simulink model "SIM_EXO_DAL"  (R2021b)
settings: Solver=VariableStepAuto  StartTime=0.0  StopTime=60  FixedStep=0.0001  RelTol=1e-4
undefined symbols (not defined in the file): b, dq, q, X, Y, Z
libraries: sm_lib x47, nesl_utility x7
(part 3 of 25)

== matlab function SIM_EXO_DAL/PID(LGR)/H_Matrix ==
  data: q input; H output
function H = H_Matrix(q)
%#codegen
q1 = q(1);
q2 = q(2);
q3 = q(3);
q4 = q(4);
q5 = q(5);
q6 = q(6);
%    This function was generated by the Symbolic Math Toolbox version 9.0.
%    02-Dec-2021 20:02:35

t2 = cos(q2);
t3 = cos(q4);
t4 = cos(q5);
t5 = cos(q6);
t6 = sin(q2);
t7 = sin(q4);
t8 = sin(q5);
t9 = sin(q6);
t10 = q1+q2;
t11 = q4.*2.0;
t12 = q5.*2.0;
t13 = q6.*2.0;
t30 = 9.007199254740992e+15;
t14 = cos(t12);
t15 = cos(t13);
t16 = t3.^2;
t17 = t4.^2;
t18 = t5.^2;
t19 = sin(t11);
t20 = sin(t12);
t21 = sin(t13);
t22 = cos(t10);
t23 = sin(t10);
t29 = t8.*5.110348748545983e-1;
t31 = t4.*t5.*5.110348748545983e-1;
t32 = t4.*t9.*5.110348748545983e-1;
t33 = t4.*t7.*8.595599785252598e-1;
t34 = t3.*t9.*8.595599785252598e-1;
t35 = t5.*1.33637579258949e-4;
t37 = t3.*t5.*8.595599785252598e-1;
t38 = t9.*7.26350610236655e-5;
t39 = t5.*t7.*t8.*8.595599785252598e-1;
t40 = t7.*t8.*t9.*8.595599785252598e-1;
t41 = t9.*1.744166498897461e-6;
t42 = t5.*1.246862701090643e-6;
t43 = t9.*1.246862701090643e-6;
t44 = t8.*4.20092050615074e-6;
t45 = t5.*3.383302988283333e-6;
t51 = t4.*t9.*3.383302988283333e-6;
t52 = t8.*1.758766830582798e-8;
t53 = t4.*t5.*1.744166498897461e-6;
t54 = t5.*t8.*8.01825475553694e-7;
t55 = t4.*t5.*(-1.246862701090643e-6);
t56 = t4.*t9.*(-1.246862701090643e-6);
t57 = t4.*2.524706033578261e-9;
t58 = t8.*t9.*4.35810366141993e-7;
t59 = t5.*3.146556677756745e-13;
t60 = t8.*3.146556677756745e-13;
t61 = t8.*4.126305279697715e-13;
t62 = t9.*4.126305279697715e-13;
t63 = t4.*t9.*3.146556677756745e-13;
t65 = t4.*t5.*4.126305279697715e-13;
t66 = t5.*t8.*8.4155913e-14;
t67 = t8.*t9.*8.4155913e-14;
t68 = (q3.*t30)./4.503599627370496e+15;
t70 = (q3.*t30)./9.007199254740992e+15;
t78 = t8.*6.829346359246847e-5;
t82 = t3.*5.316841594276996e-5;
t83 = t4.*6.932317328700695e-5;
t84 = t3.*1.166014850920627e-4;
t85 = t3.*t5.*1.148695147579899e-4;
t86 = t8.*3.161026044296245e-5;
t87 = t4.*t9.*6.829346359246847e-5;
t88 = t4.*t7.*1.148695147579899e-4;
t89 = t8.*3.711904932028501e-5;
t90 = t8.*2.146816885134859e-6;
t91 = t8.*3.004073648334264e-7;
t93 = t4.*3.726186752973823e-7;
t94 = t8.*3.726186752973823e-7;
t95 = t4.*t7.*5.316841594276996e-5;
t97 = t4.*3.60334715805357e-7;
t98 = t8.*3.60334715805357e-7;
t99 = t4.*1.153569201933121e-6;
t100 = t7.*t8.*1.166014850920627e-4;
t101 = t3.*2.28624364216682e-6;
t102 = t8.*8.987911871652987e-9;
t103 = t4.*t5.*3.711904932028501e-5;
t104 = t7.*t8.*t9.*1.148695147579899e-4;
t106 = t4.*t7.*6.243419149368285e-5;
t107 = t3.*t9.*6.243419149368285e-5;
t108 = t4.*t5.*8.913299084896471e-7;
t115 = t4.*t9.*1.728985819212562e-6;
t116 = t4.*t5.*6.371903244127231e-7;
t117 = t4.*t9.*6.371903244127231e-7;
t118 = t7.*t8.*1.940301860461398e-6;
t119 = t4.*t7.*3.610943140053254e-6;
t120 = t3.*t5.*2.908151843953269e-6;
t122 = t4.*t7.*5.052847873416058e-7;
t123 = t3.*t5.*1.07175327657342e-6;
t124 = t3.*t9.*1.07175327657342e-6;
t125 = t3.*t9.*1.49921571833678e-6;
t126 = t4.*t7.*6.267441153167058e-7;
t127 = t7.*t8.*6.267441153167058e-7;
t128 = t3.*1.511765579126689e-8;
t129 = t4.*t7.*6.060825118201251e-7;
t131 = t7.*t8.*6.060825118201251e-7;
t134 = t4.*1.290212831914316e-9;
t135 = t8.*1.608000198040319e-13;
t137 = t3.*2.170136264005124e-9;
t140 = t5.*t7.*t8.*6.243419149368285e-5;
t141 = t3.*t4.*t9.*6.892170885479394e-7;
t143 = t7.*t8.*t9.*2.908151843953269e-6;
t144 = t5.*t7.*t8.*1.07175327657342e-6;
t146 = t7.*t8.*t9.*1.07175327657342e-6;
t147 = t5.*t7.*t8.*1.49921571833678e-6;
t149 = t4.*t7.*1.511765579126689e-8;
t150 = t4.*t9.*1.608000198040319e-13;
t153 = t7.*t8.*2.170136264005124e-9;
t154 = t3.*t8.*(-1.511765579126689e-8);
t157 = t3.*t4.*t5.*3.746051489620971e-7;
t158 = t4.*t5.*7.16776774470491e-12;
t159 = t4.*t9.*7.16776774470491e-12;
t160 = t8.*2.10868590222219e-13;
t161 = t3.*t5.*2.7046541903611e-13;
t162 = t4.*t7.*2.7046541903611e-13;
t164 = t3.*t5.*1.205617579517561e-11;
t165 = t3.*t9.*1.205617579517561e-11;
t167 = t4.*t7.*3.546806877605634e-13;
t168 = t3.*t9.*3.546806877605634e-13;
t169 = t4.*t5.*2.10868590222219e-13;
t172 = t7.*t8.*t9.*2.7046541903611e-13;
t173 = t5.*t7.*t8.*1.205617579517561e-11;
t174 = t7.*t8.*t9.*1.205617579517561e-11;
t177 = t5.*t7.*t8.*3.546806877605634e-13;
t180 = t3.*t8.*t9.*(-3.546806877605634e-13);
t192 = t3.*2.625549359694895e-3;
t193 = t4.*1.560969940408669e-3;
t194 = t8.*1.560969940408669e-3;
t195 = t6.*t8.*1.324388487819695e-2;
t196 = t2.*t8.*5.463144604697158e-2;
t202 = t4.*t7.*2.625549359694895e-3;
t204 = t7.*t8.*2.625549359694895e-3;
t207 = t4.*t6.*t7.*2.227619671697157e-2;
t208 = t7.*5.363539617571206e-4;
t209 = t3.*t5.*(-2.625549359694895e-3);
t210 = t4.*t5.*(-1.560969940408669e-3);
t211 = t4.*t9.*(-1.560969940408669e-3);
t217 = t2.*t4.*t7.*9.189001945180305e-2;
t218 = t5.*1.184846851663018e-6;
t223 = t7.*3.050168925520967e-6;
t226 = t7.*6.689201101650821e-6;
t230 = t3.*t4.*5.363539617571206e-4;
t231 = t3.*t8.*5.363539617571206e-4;
t233 = t3.*t9.*6.589841321991422e-6;
t237 = t3.*t4.*3.050168925520967e-6;
t240 = t3.*t8.*6.689201101650821e-6;
t246 = t3.*t8.*1.545129867076994e-8;
t247 = t3.*t4.*t9.*7.044279371874937e-7;
t248 = t9.*6.439911875946239e-7;
t249 = t3.*t5.*3.581728501918121e-6;
t255 = t5.*t7.*t8.*6.589841321991422e-6;
t269 = t3.*t7.*t8.*t9.*4.188040994443703e-7;
t270 = t3.*2.783427048984746e-6;
t271 = t4.*t5.*t7.*t8.*1.408855874374987e-6;
t272 = t3.*t4.*t5.*t9.*1.440030993265091e-6;
t273 = t7.*t8.*t9.*3.581728501918121e-6;
t275 = t3.*t4.*t7.*9.186272837068685e-9;
t280 = t3.*t4.*3.476977846858022e-8;
t281 = t3.*t8.*3.476977846858022e-8;
t282 = t3.*t4.*t5.*3.828725908394669e-7;
t286 = t3.*t5.*t7.*t8.*t9.*8.561427670149984e-7;
t294 = t3.*t5.*t7.*t8.*2.276295446893622e-7;
t302 = t7.*t8.*5.200343311959535e-6;
t303 = t7.*t9.*2.764345231392299e-13;
t306 = t4.*t5.*t7.*t8.*t9.*2.190813206274814e-6;
t308 = t3.*t4.*1.093188572509221e-6;
t311 = t4.*t7.*t8.*t9.*7.657451816789338e-7;
t320 = t3.*t5.*t8.*2.764345231392299e-13;
t328 = t4.*t8.*t9.*3.006136635626675e-13;
t332 = t5.*t7.*3.625084017661248e-13;
t335 = t3.*t7.*t8.*6.499342678834474e-7;
t341 = t3.*t4.*t5.*t7.*1.643488359943407e-13;
t345 = t3.*t8.*t9.*3.625084017661248e-13;
t346 = t4.*t7.*t8.*5.185406908527248e-7;
t348 = t4.*t5.*t8.*3.94216241479634e-13;
t350 = t3.*t4.*t7.*t9.*2.155224072299545e-13;
t360 = t4.*t7.*6.689200410011394e-6;
t379 = t8.*2.086042441322004e-7;
t384 = t8.*1.133811468776912e-7;
t386 = t4.*t9.*2.086042441322004e-7;
t388 = t2.*t4.*t5.*1.769880715106441e-6;
t389 = t4.*t6.*t9.*1.769880715106441e-6;
t390 = t5.*t6.*t8.*1.769880715106441e-6;
t391 = t3.*4.911624408131596e-10;
t392 = t4.*t5.*1.133811468776912e-7;
t394 = t3.*t5.*3.508720606545093e-7;
t397 = t4.*t7.*3.508720606545093e-7;
t398 = t7.*t9.*3.508720606545093e-7;
t399 = t2.*t7.*4.167215943261981e-9;
t400 = t3.*t6.*4.167215943261981e-9;
t401 = t6.*t7.*t9.*2.976937004352228e-6;
t402 = t4.*t5.*1.209061939415321e-5;
t405 = t2.*t4.*t9.*7.30081420113316e-6;
t406 = t2.*t5.*t8.*7.30081420113316e-6;
t407 = t4.*t5.*t6.*7.30081420113316e-6;
t410 = t2.*t3.*t9.*2.976937004352228e-6;
t411 = t3.*t5.*t6.*2.976937004352228e-6;
t414 = t8.*1.646190906295504e-7;
t415 = t2.*t3.*t5.*1.22799597575967e-5;
t417 = t2.*t7.*t9.*1.22799597575967e-5;
t418 = t3.*t6.*t9.*1.22799597575967e-5;
t422 = t3.*t9.*2.033640570959539e-5;
t423 = t4.*t7.*1.907069379620846e-7;
t424 = t3.*t9.*1.907069379620846e-7;
t425 = t5.*t7.*1.907069379620846e-7;
t428 = t6.*t8.*t9.*9.619703863182361e-7;
t429 = t2.*t4.*1.396693317797299e-6;
t430 = t6.*t8.*1.396693317797299e-6;
t431 = t2.*t4.*t5.*3.96815841743287e-6;
t432 = t2.*t8.*t9.*3.96815841743287e-6;
t433 = t4.*t6.*t9.*3.96815841743287e-6;
t434 = t2.*t3.*t5.*1.618032907912407e-6;
t437 = t2.*t3.*1.718989821069714e-8;
t438 = t3.*t6.*t9.*1.618032907912407e-6;
t439 = t5.*t6.*t7.*1.618032907912407e-6;
t440 = t6.*t7.*1.718989821069714e-8;
t441 = t7.*t8.*t9.*(-3.508720606545093e-7);
t443 = t2.*t5.*t7.*t8.*2.976937004352228e-6;
t445 = t4.*t5.*t6.*t7.*2.976937004352228e-6;
t446 = t2.*t4.*t9.*9.619703863182361e-7;
t447 = t4.*t5.*t6.*9.619703863182361e-7;
t449 = t4.*t9.*6.571526380364474e-6;
t451 = t3.*t5.*1.105329861487718e-5;
t453 = t2.*t4.*t5.*t7.*1.22799597575967e-5;
t457 = t5.*t6.*t7.*t8.*1.22799597575967e-5;
t461 = t7.*4.452917654948397e-7;
t462 = t5.*t7.*t8.*2.033640570959539e-5;
t466 = t2.*t8.*5.761404326386517e-6;
t467 = t4.*t6.*5.761404326386517e-6;
t469 = t3.*t5.*t6.*t8.*(-2.976937004352228e-6);
t471 = t2.*t3.*t9.*6.674437170347525e-6;
t472 = t2.*t5.*t7.*6.674437170347525e-6;
t473 = t3.*t5.*t6.*6.674437170347525e-6;
t474 = t4.*9.541257312828922e-6;
t476 = t3.*t8.*2.768890910755245e-7;
t477 = t4.*t7.*2.768890910755245e-7;
t478 = t2.*t3.*3.778031034908185e-6;
t479 = t2.*t7.*t8.*t9.*(-1.22799597575967e-5);
t481 = t6.*t7.*3.778031034908185e-6;
t482 = t2.*t7.*t8.*t9.*1.618032907912407e-6;
t484 = t4.*t6.*t7.*t9.*1.618032907912407e-6;
t488 = t7.*t8.*t9.*1.105329861487718e-5;
t490 = t2.*t7.*t8.*2.349236299369594e-6;
t491 = t3.*t6.*t8.*2.349236299369594e-6;
t492 = t4.*t6.*t7.*2.349236299369594e-6;
t494 = t3.*t6.*t8.*t9.*(-1.618032907912407e-6);
t496 = t5.*t6.*t7.*t8.*(-1.618032907912407e-6);
t497 = t2.*t7.*1.558449809444963e-5;
t498 = t3.*t6.*1.558449809444963e-5;
t500 = t2.*t4.*t7.*t9.*6.674437170347525e-6;
t502 = t6.*t7.*t8.*t9.*6.674437170347525e-6;
t503 = t3.*2.010604972694953e-5;
t511 = t4.*t5.*2.189414175010785e-14;
t512 = t4.*t9.*2.189414175010785e-14;
t513 = t7.*t8.*1.604838208596364e-5;
t514 = t2.*t3.*t8.*9.690674399615435e-6;
t515 = t2.*t4.*t7.*9.690674399615435e-6;
t516 = t6.*t7.*t8.*9.690674399615435e-6;
t517 = t7.*6.664488561844862e-7;
t519 = t3.*t5.*3.682591724861488e-14;
t521 = t3.*t9.*3.682591724861488e-14;
t524 = t5.*t7.*t8.*3.682591724861488e-14;
t525 = t7.*t8.*t9.*3.682591724861488e-14;
t526 = t4.*2.11749498538388e-7;
t534 = t2.*t8.*1.796566294495167e-6;
t535 = t4.*t6.*1.796566294495167e-6;
t539 = t2.*t4.*7.410893064247368e-6;
t540 = t6.*t8.*7.410893064247368e-6;
t542 = t3.*t4.*3.561623743745041e-7;
t543 = t7.*t8.*3.561623743745041e-7;
t544 = t8.*1.227291709418896e-5;
t545 = t2.*t4.*t7.*3.021822113324163e-6;
t546 = t3.*t4.*t6.*3.021822113324163e-6;
t547 = t6.*t7.*t8.*3.021822113324163e-6;
t553 = t4.*t7.*2.06430301981345e-5;
t556 = t2.*t3.*t4.*1.246511225866906e-5;
t557 = t2.*t7.*t8.*1.246511225866906e-5;
t558 = t4.*t6.*t7.*1.246511225866906e-5;
t593 = t2.*1.410504133294943e-4;
t596 = t6.*4.897880306001738e-4;
t24 = t23.*7.742227997977903e+15;
t25 = t22.*4.602992943936994e+15;
t26 = t23.*4.602992943936994e+15;
t27 = t22.*7.742227997977903e+15;
t36 = -t31;
t46 = -t40;
t48 = t4.*t42;
t49 = t4.*t43;
t64 = -t62;
t69 = sin(t68);
t71 = cos(t70);
t72 = sin(t70);
t92 = -t83;
t96 = -t90;
t105 = -t93;
t109 = -t97;
t110 = -t98;
t111 = -t99;
t112 = -t102;
t113 = -t103;
t114 = -t104;
t121 = t29+t33;
t130 = -t116;
t132 = -t117;
t133 = -t119;
t136 = -t123;
t138 = -t125;
t139 = -t128;
t142 = -t129;
t145 = -t134;
t148 = t8.*t128;
t151 = -t143;
t152 = -t147;
t155 = -t149;
t156 = -t150;
t163 = -t157;
t166 = -t161;
t170 = -t165;
t171 = t8.*t161;
t175 = -t169;
t176 = t8.*t168;
t178 = -t173;
t179 = -t174;
t181 = t52+t57;
t182 = t20.*3.726186322907759e-7;
t197 = -t193;
t200 = -t195;
t201 = t5.*t192;
t203 = t9.*t192;
t205 = t5.*t193;
t206 = t9.*t193;
t219 = -t207;
t221 = t5.*t204;
t222 = t9.*t204;
t224 = t18.*4.280713835074992e-7;
t229 = t21.*3.256264776948168e-7;
t251 = t5.*t16.*4.188040994443703e-7;
t253 = t5.*t17.*7.660427522186475e-7;
t257 = t9.*t16.*2.276295446893622e-7;
t258 = t16.*t18.*8.561427670149984e-7;
t260 = t19.*4.420145378913349e-10;
t261 = -t247;
t262 = -t249;
t268 = t5.*t9.*t16.*1.302505910779267e-6;
t276 = t17.*t18.*7.829937223708732e-7;
t277 = t5.*t9.*t17.*1.191219491402018e-6;
t278 = t3.*t4.*t18.*2.190813206274814e-6;
t287 = -t269;
t288 = -t270;
t289 = -t271;
t290 = t9.*t17.*4.163616429052617e-7;
t291 = -t272;
t292 = -t275;
t297 = -t281;
t298 = t3.*t7.*t8.*t18.*1.302505910779267e-6;
t305 = -t286;
t309 = t4.*t7.*t8.*t18.*1.440030993265091e-6;
t315 = -t306;
t316 = -t308;
t321 = -t311;
t322 = t5.*t16.*t17.*(-4.188040994443703e-7);
t324 = t5.*t9.*t16.*t17.*6.512529553896337e-7;
t325 = t16.*1.035461175802946e-6;
t326 = t9.*t16.*t17.*(-2.276295446893622e-7);
t327 = t16.*t17.*t18.*(-4.280713835074992e-7);
t329 = t17.*2.81948171692439e-7;
t331 = -t320;
t338 = t7.*t9.*t17.*5.528690462784599e-13;
t343 = -t335;
t347 = t4.*t8.*t9.*t16.*1.643488359943407e-13;
t349 = t16.*t17.*1.54144203823673e-7;
t351 = -t350;
t352 = t5.*t7.*t17.*7.250168035322496e-13;
t353 = t4.*t5.*t8.*t16.*2.155224072299545e-13;
t355 = t35+t38+4.36041e-5;
t362 = -t360;
t363 = t20.*3.483029800032151e-7;
t364 = t43+t45+8.01825475553694e-7;
t365 = t7.*t17.*1.281152254279884e-6;
t368 = t41+t42+4.35810366141993e-7;
t371 = t4.*t8.*t16.*3.808422322424164e-7;
t387 = t5.*t379;
t393 = t9.*t384;
t395 = -t389;
t396 = -t390;
t404 = -t392;
t409 = -t398;
t412 = -t399;
t413 = -t400;
t419 = t8.*t394;
t420 = t5.*t397;
t421 = t8.*t398;
t426 = -t410;
t427 = -t411;
t435 = -t417;
t436 = -t418;
t442 = -t422;
t444 = t8.*t411;
t448 = t8.*t401;
t450 = -t428;
t452 = t8.*t415;
t454 = -t430;
t455 = -t431;
t456 = t8.*t417;
t458 = -t438;
t459 = -t439;
t460 = -t440;
t463 = t8.*t424;
t464 = t9.*t423;
t465 = t8.*t425;
t468 = -t443;
t470 = -t445;
t480 = -t457;
t483 = t8.*t438;
t485 = t8.*t439;
t486 = -t462;
t489 = -t481;
t493 = -t482;
t495 = -t484;
t499 = t8.*t471;
t501 = t8.*t472;
t505 = -t488;
t506 = -t490;
t507 = -t491;
t508 = -t492;
t509 = -t502;
t518 = -t513;
t520 = -t516;
t522 = -t517;
t523 = -t521;
t531 = -t524;
t532 = -t525;
t533 = -t526;
t541 = -t539;
t548 = -t542;
t554 = -t547;
t560 = -t556;
t712 = t51+t55+t60+t67;
t736 = t53+t56+t61+t66;
t1090 = t44+t54+t58+t63+t65;
t28 = -t26;
t47 = t24+t25;
t73 = t71.^2;
t74 = t3.*t71;
t75 = t7.*t71;
t76 = t71-1.0;
t183 = t71.*2.118754404193375e+31;
t184 = -t182;
t186 = t59+t64;
t189 = t4.*t71.*5.157359871151559e-3;
t232 = -t224;
t234 = -t229;
t267 = -t253;
t295 = -t276;
t296 = -t277;
t307 = -t290;
t312 = t17.*t251;
t317 = t17.*t257;
t318 = t16.*t17.*t224;
t319 = -t309;
t336 = -t324;
t337 = -t325;
t340 = t3.*t30.*t72.*4.602992943936994e+15;
t344 = -t338;
t354 = -t352;
t356 = t34+t36+t39;
t357 = t32+t37+t46;
t361 = t3.*t8.*t30.*t72.*6.661338147750939e-19;
t366 = -t363;
t369 = t71.*7.38843356682345e-1;
t370 = t71.*2.61156643317655e-1;
t372 = t71.*4.392651260556773e-1;
t373 = t71.*4.931128922368695e-2;
t374 = -t371;
t377 = t30.*t72.*8.001214128951626e+33;
t381 = t4.*t30.*t72.*8.368294830410569e+32;
t382 = t7.*t8.*t30.*t72.*4.97520895370488e+32;
t383 = t4.*t71.*1.511765579126689e-8;
t403 = t4.*t16.*t71.*3.023531158253378e-8;
t408 = t16.*t71.*2.909656073620116e-9;
t487 = -t7.*t30.*t72.*(t26-t27);
t510 = t7.*t30.*t72.*(t26-t27);
t527 = t3.*t30.*t72.*5.673626844500105e-17;
t528 = t7.*t30.*t72.*5.673626844500105e-17;
t529 = t4.*t30.*t72.*9.543032792050485e-17;
t530 = t8.*t30.*t72.*9.543032792050485e-17;
t538 = t3.*t30.*t72.*3.404176106700063e-19;
t549 = t5.*t8.*t30.*t72.*5.725819675230291e-19;
t550 = t8.*t9.*t30.*t72.*5.725819675230291e-19;
t551 = t4.*t5.*t7.*t30.*t72.*3.404176106700063e-19;
t552 = t4.*t7.*t9.*t30.*t72.*3.404176106700063e-19;
t561 = t2.*t8.*t71.*2.227619671697157e-2;
t562 = t4.*t71.*5.088811214040866e-2;
t563 = t8.*t71.*5.088811214040866e-2;
t565 = t6.*t8.*t71.*9.189001945180305e-2;
t588 = t2.*t71.*4.472183499114333e-13;
t603 = t6.*t71.*1.844789907123413e-12;
t614 = t71.*1.454432002254732e-9;
t653 = t3.*t30.*t72.*(t26-t27).*(-1.232595164407831e-32);
t666 = t7.*t30.*t72.*9.827649182848514e-18;
H = ft_1({t100,t101,t102,t105,t106,t107,t108,t109,t1090,t110,t111,t112,t113,t114,t115,t118,t119,t120,t121,t122,t124,t126,t127,t130,t131,t132,t133,t134,t135,t136,t137,t138,t139,t14,t140,t141,t142,t144,t145,t146,t149,t15,t150,t151,t152,t153,t154,t155,t156,t158,t159,t16,t160,t161,t162,t163,t164,t166,t167,t168,t169,t17,t170,t171,t172,t175,t177,t178,t179,t18,t180,t181,t183,t184,t186,t189,t19,t192,t194,t196,t197,t2,t20,t200,t202,t203,t204,t208,t209,t21,t210,t211,t217,t218,t219,t22,t221,t222,t223,t226,t23,t230,t231,t232,t233,t234,t237,t240,t246,t247,t248,t251,t253,t255,t257,t258,t26,t260,t261,t262,t267,t268,t27,t271,t272,t273,t276,t277,t278,t28,t280,t282,t287,t288,t289,t290,t291,t292,t294,t295,t296,t297,t298,t3,t30,t302,t303,t305,t306,t307,t308,t309,t311,t315,t316,t319,t320,t321,t322,t326,t327,t328,t329,t331,t332,t336,t337,t338,t340,t341,t343,t344,t345,t346,t347,t348,t349,t35,t351,t352,t353,t354,t355,t356,t357,t361,t362,t364,t365,t366,t368,t369,t370,t372,t373,t374,t377,t379,t38,t381,t382,t383,t384,t386,t387,t388,t390,t391,t393,t394,t395,t396,t397,t4,t401,t402,t403,t404,t405,t406,t407,t408,t409,t41,t412,t413,t414,t415,t419,t42,t420,t423,t424,t425,t426,t427,t428,t429,t43,t430,t432,t433,t434,t435,t436,t437,t441,t442,t446,t447,t448,t449,t45,t450,t451,t452,t453,t454,t455,t458,t459,t460,t461,t463,t464,t465,t466,t467,t468,t469,t47,t470,t471,t472,t473,t474,t476,t477,t478,t479,t480,t486,t489,t493,t494,t495,t496,t497,t498,t499,t5,t500,t501,t503,t505,t506,t507,t508,t509,t510,t511,t512,t514,t515,t518,t519,t52,t520,t521,t522,t523,t524,t527,t528,t529,t530,t531,t532,t533,t534,t535,t538,t539,t540,t541,t543,t544,t545,t546,t548,t549,t550,t551,t552,t553,t554,t557,t558,t560,t561,t562,t563,t565,t588,t59,t593,t596,t6,t603,t61,t614,t62,t653,t666,t69,t7,t71,t712,t72,t73,t736,t74,t75,t76,t78,t8,t82,t84,t85,t86,t87,t88,t89,t9,t90,t91,t92,t94,t95,t96});
end
function H = ft_1(ct)
t100 = ct{1};
t101 = ct{2};
t102 = ct{3};
t105 = ct{4};
t106 = ct{5};
t107 = ct{6};
t108 = ct{7};
t109 = ct{8};
t1090 = ct{9};
t110 = ct{10};
t111 = ct{11};
t112 = ct{12};
t113 = ct{13};
t114 = ct{14};
t115 = ct{15};
t118 = ct{16};
t119 = ct{17};
t120 = ct{18};
t121 = ct{19};
t122 = ct{20};
t124 = ct{21};
t126 = ct{22};
t127 = ct{23};
t130 = ct{24};
t131 = ct{25};
t132 = ct{26};
t133 = ct{27};
t134 = ct{28};
t135 = ct{29};
t136 = ct{30};
t137 = ct{31};
t138 = ct{32};
t139 = ct{33};
t14 = ct{34};
t140 = ct{35};
t141 = ct{36};
t142 = ct{37};
t144 = ct{38};
t145 = ct{39};
t146 = ct{40};
t149 = ct{41};
t15 = ct{42};
t150 = ct{43};
t151 = ct{44};
t152 = ct{45};
t153 = ct{46};
t154 = ct{47};
t155 = ct{48};
t156 = ct{49};
t158 = ct{50};
t159 = ct{51};
t16 = ct{52};
t160 = ct{53};
t161 = ct{54};
t162 = ct{55};
t163 = ct{56};
t164 = ct{57};
t166 = ct{58};
t167 = ct{59};
t168 = ct{60};
t169 = ct{61};
t17 = ct{62};
t170 = ct{63};
t171 = ct{64};
t172 = ct{65};
t175 = ct{66};
t177 = ct{67};
t178 = ct{68};
t179 = ct{69};
t18 = ct{70};
t180 = ct{71};
t181 = ct{72};
t183 = ct{73};
t184 = ct{74};
t186 = ct{75};
t189 = ct{76};
t19 = ct{77};
t192 = ct{78};
t194 = ct{79};
t196 = ct{80};
t197 = ct{81};
t2 = ct{82};
t20 = ct{83};
t200 = ct{84};
t202 = ct{85};
t203 = ct{86};
t204 = ct{87};
t208 = ct{88};
t209 = ct{89};
t21 = ct{90};
t210 = ct{91};
t211 = ct{92};
t217 = ct{93};
t218 = ct{94};
t219 = ct{95};
t22 = ct{96};
t221 = ct{97};
t222 = ct{98};
t223 = ct{99};
t226 = ct{100};
t23 = ct{101};
t230 = ct{102};
t231 = ct{103};
t232 = ct{104};
t233 = ct{105};
t234 = ct{106};
t237 = ct{107};
t240 = ct{108};
t246 = ct{109};
t247 = ct{110};
t248 = ct{111};
t251 = ct{112};
t253 = ct{113};
t255 = ct{114};
t257 = ct{115};
t258 = ct{116};
t26 = ct{117};
t260 = ct{118};
t261 = ct{119};
t262 = ct{120};
t267 = ct{121};
t268 = ct{122};
t27 = ct{123};
t271 = ct{124};
t272 = ct{125};
t273 = ct{126};
t276 = ct{127};
t277 = ct{128};
t278 = ct{129};
t28 = ct{130};
t280 = ct{131};
t282 = ct{132};
t287 = ct{133};
t288 = ct{134};
t289 = ct{135};
t290 = ct{136};
t291 = ct{137};
t292 = ct{138};
t294 = ct{139};
t295 = ct{140};
t296 = ct{141};
t297 = ct{142};
t298 = ct{143};
t3 = ct{144};
t30 = ct{145};
t302 = ct{146};
t303 = ct{147};
t305 = ct{148};
t306 = ct{149};
t307 = ct{150};
t308 = ct{151};
t309 = ct{152};
t311 = ct{153};
t315 = ct{154};
t316 = ct{155};
t319 = ct{156};
t320 = ct{157};
t321 = ct{158};
t322 = ct{159};
t326 = ct{160};
t327 = ct{161};
t328 = ct{162};
t329 = ct{163};
t331 = ct{164};
t332 = ct{165};
t336 = ct{166};
t337 = ct{167};
t338 = ct{168};
t340 = ct{169};
t341 = ct{170};
t343 = ct{171};
t344 = ct{172};
t345 = ct{173};
t346 = ct{174};
t347 = ct{175};
t348 = ct{176};
t349 = ct{177};
t35 = ct{178};
t351 = ct{179};
t352 = ct{180};
t353 = ct{181};
t354 = ct{182};
t355 = ct{183};
t356 = ct{184};
t357 = ct{185};
t361 = ct{186};
t362 = ct{187};
t364 = ct{188};
t365 = ct{189};
t366 = ct{190};
t368 = ct{191};
t369 = ct{192};
t370 = ct{193};
t372 = ct{194};
t373 = ct{195};
t374 = ct{196};
t377 = ct{197};
t379 = ct{198};
t38 = ct{199};
t381 = ct{200};
t382 = ct{201};
t383 = ct{202};
t384 = ct{203};
t386 = ct{204};
t387 = ct{205};
t388 = ct{206};
t390 = ct{207};
t391 = ct{208};
t393 = ct{209};
t394 = ct{210};
t395 = ct{211};
t396 = ct{212};
t397 = ct{213};
t4 = ct{214};
t401 = ct{215};
t402 = ct{216};
t403 = ct{217};
t404 = ct{218};
t405 = ct{219};
t406 = ct{220};
t407 = ct{221};
t408 = ct{222};
t409 = ct{223};
t41 = ct{224};
t412 = ct{225};
t413 = ct{226};
t414 = ct{227};
t415 = ct{228};
t419 = ct{229};
t42 = ct{230};
t420 = ct{231};
t423 = ct{232};
t424 = ct{233};
t425 = ct{234};
t426 = ct{235};
t427 = ct{236};
t428 = ct{237};
t429 = ct{238};
t43 = ct{239};
t430 = ct{240};
t432 = ct{241};
t433 = ct{242};
t434 = ct{243};
t435 = ct{244};
t436 = ct{245};
t437 = ct{246};
t441 = ct{247};
t442 = ct{248};
t446 = ct{249};
t447 = ct{250};
t448 = ct{251};
t449 = ct{252};
t45 = ct{253};
t450 = ct{254};
t451 = ct{255};
t452 = ct{256};
t453 = ct{257};
t454 = ct{258};
t455 = ct{259};
t458 = ct{260};
t459 = ct{261};
t460 = ct{262};
t461 = ct{263};
t463 = ct{264};
t464 = ct{265};
t465 = ct{266};
t466 = ct{267};
t467 = ct{268};
t468 = ct{269};
t469 = ct{270};
t47 = ct{271};
t470 = ct{272};
t471 = ct{273};
t472 = ct{274};
t473 = ct{275};
t474 = ct{276};
t476 = ct{277};
t477 = ct{278};
t478 = ct{279};
t479 = ct{280};
t480 = ct{281};
t486 = ct{282};
t489 = ct{283};
t493 = ct{284};
t494 = ct{285};
t495 = ct{286};
t496 = ct{287};
t497 = ct{288};
t498 = ct{289};
t499 = ct{290};
t5 = ct{291};
t500 = ct{292};
t501 = ct{293};
t503 = ct{294};
t505 = ct{295};
t506 = ct{296};
t507 = ct{297};
t508 = ct{298};
t509 = ct{299};
t510 = ct{300};
t511 = ct{301};
t512 = ct{302};
t514 = ct{303};
t515 = ct{304};
t518 = ct{305};
t519 = ct{306};
t52 = ct{307};
t520 = ct{308};
t521 = ct{309};
t522 = ct{310};
t523 = ct{311};
t524 = ct{312};
t527 = ct{313};
t528 = ct{314};
t529 = ct{315};
t530 = ct{316};
t531 = ct{317};
t532 = ct{318};
t533 = ct{319};
t534 = ct{320};
t535 = ct{321};
t538 = ct{322};
t539 = ct{323};
t540 = ct{324};
t541 = ct{325};
t543 = ct{326};
t544 = ct{327};
t545 = ct{328};
t546 = ct{329};
t548 = ct{330};
t549 = ct{331};
t550 = ct{332};
t551 = ct{333};
t552 = ct{334};
t553 = ct{335};
t554 = ct{336};
t557 = ct{337};
t558 = ct{338};
t560 = ct{339};
t561 = ct{340};
t562 = ct{341};
t563 = ct{342};
t565 = ct{343};
t588 = ct{344};
t59 = ct{345};
t593 = ct{346};
t596 = ct{347};
t6 = ct{348};
t603 = ct{349};
t61 = ct{350};
t614 = ct{351};
t62 = ct{352};
t653 = ct{353};
t666 = ct{354};
t69 = ct{355};
t7 = ct{356};
t71 = ct{357};
t712 = ct{358};
t72 = ct{359};
t73 = ct{360};
t736 = ct{361};
t74 = ct{362};
t75 = ct{363};
t76 = ct{364};
t78 = ct{365};
t8 = ct{366};
t82 = ct{367};
t84 = ct{368};
t85 = ct{369};
t86 = ct{370};
t87 = ct{371};
t88 = ct{372};
t89 = ct{373};
t9 = ct{374};
t90 = ct{375};
t91 = ct{376};
t92 = ct{377};
t94 = ct{378};
t95 = ct{379};
t96 = ct{380};
t668 = t8.*t30.*t72.*4.008952214699383e-22;
t670 = t2.*t3.*t4.*t30.*t72.*2.877233365226343e-18;
t671 = t3.*t30.*t72.*4.549258542705501e-23;
t672 = t3.*t4.*t6.*t30.*t72.*1.186867907736671e-17;
t674 = t3.*t4.*t30.*t72.*9.827649182848514e-18;
t676 = t3.*t8.*t30.*t72.*9.827649182848514e-18;
t679 = t5.*t30.*t72.*1.530369361342075e-22;
t681 = t7.*t9.*t30.*t72.*(-9.827649182848514e-18);
t682 = t3.*t5.*t30.*t72.*9.098517085411002e-23;
t685 = t3.*t30.*t72.*2.472625392454631e-23;
t686 = t3.*t5.*t9.*t30.*t72.*1.414846738462756e-22;
t687 = t8.*t30.*t72.*1.678396953782234e-24;
t688 = t3.*t9.*t30.*t72.*4.945250784909262e-23;
t689 = t9.*t30.*t72.*8.317905230417136e-23;
t691 = t4.*t5.*t7.*t30.*t72.*4.549258542705501e-23;
t692 = t7.*t8.*t9.*t30.*t72.*4.549258542705501e-23;
t693 = t3.*t18.*t30.*t72.*9.299848787979342e-23;
t694 = t4.*t9.*t30.*t72.*7.651846806710377e-23;
t695 = t5.*t8.*t30.*t72.*7.651846806710377e-23;
t696 = t3.*t8.*t30.*t72.*9.978586703210931e-25;
t697 = t4.*t7.*t30.*t72.*9.978586703210931e-25;
t700 = t4.*t18.*t30.*t72.*2.379770328738529e-22;
t701 = t3.*t4.*t9.*t30.*t72.*(-4.549258542705501e-23);
t705 = t4.*t5.*t9.*t30.*t72.*1.564233326885588e-22;
t707 = t5.*t17.*t30.*t72.*(-1.530369361342075e-22);
t708 = t3.*t4.*t5.*t9.*t30.*t72.*9.299848787979342e-23;
t709 = t5.*t7.*t8.*t9.*t30.*t72.*9.299848787979342e-23;
t710 = t4.*t5.*t30.*t72.*4.158952615208568e-23;
t711 = t8.*t9.*t30.*t72.*4.158952615208568e-23;
t713 = t4.*t5.*t7.*t8.*t30.*t72.*9.098517085411002e-23;
t714 = t3.*t4.*t18.*t30.*t72.*1.414846738462756e-22;
t715 = t7.*t8.*t18.*t30.*t72.*1.414846738462756e-22;
t717 = t7.*t9.*t30.*t72.*1.785238843466173e-29;
t720 = t8.*t30.*t72.*3.002769355787804e-29;
t722 = t4.*t7.*t9.*t30.*t72.*2.472625392454631e-23;
t723 = t5.*t7.*t8.*t30.*t72.*2.472625392454631e-23;
t724 = t5.*t9.*t17.*t30.*t72.*2.379770328738529e-22;
t726 = t17.*t18.*t30.*t72.*1.564233326885588e-22;
t727 = t4.*t5.*t7.*t8.*t9.*t30.*t72.*1.414846738462756e-22;
t729 = t4.*t7.*t8.*t9.*t30.*t72.*4.945250784909262e-23;
t732 = t4.*t7.*t8.*t18.*t30.*t72.*9.299848787979342e-23;
t733 = t4.*t30.*t72.*1.187475829122392e-22;
t735 = t3.*t4.*t30.*t72.*7.059909452387201e-23;
t738 = t7.*t8.*t30.*t72.*7.059909452387201e-23;
t744 = t30.*t72.*8.730562784510963e-22;
t748 = t9.*t17.*t30.*t72.*(-8.317905230417136e-23);
t749 = t3.*t5.*t8.*t30.*t72.*1.785238843466173e-29;
t750 = t4.*t5.*t7.*t30.*t72.*1.785238843466173e-29;
t752 = t8.*t30.*t72.*3.937746659416635e-29;
t753 = t4.*t8.*t9.*t30.*t72.*6.005538711575609e-29;
t754 = t5.*t8.*t30.*t72.*(-3.002769355787804e-29);
t755 = t30.*t69.*9.59842590807046e-26;
t758 = t17.*t30.*t72.*5.632647031707275e-23;
t760 = t3.*t30.*t72.*2.647073057000717e-22;
t761 = t4.*t5.*t71.*7.017441213090186e-7;
t764 = t7.*t9.*t17.*t30.*t72.*3.570477686932346e-29;
t766 = t5.*t7.*t30.*t72.*2.341111640349547e-29;
t772 = t4.*t7.*t8.*t30.*t72.*3.34878210114812e-23;
t773 = t8.*t71.*6.800564119502148e-6;
t780 = t4.*t9.*t71.*3.814138759241691e-7;
t782 = t2.*t4.*t9.*t71.*2.976937004352228e-6;
t783 = t2.*t5.*t8.*t71.*2.976937004352228e-6;
t784 = t4.*t5.*t6.*t71.*2.976937004352228e-6;
t785 = t5.*t8.*t30.*t72.*8.031026374039477e-30;
t786 = t8.*t9.*t30.*t72.*8.031026374039477e-30;
t789 = t4.*t5.*t8.*t30.*t72.*7.875493318833269e-29;
t791 = t3.*t8.*t9.*t30.*t72.*2.341111640349547e-29;
t792 = t4.*t7.*t9.*t30.*t72.*2.341111640349547e-29;
t798 = t8.*t71.*3.696261130697717e-6;
t799 = t5.*t7.*t17.*t30.*t72.*4.682223280699094e-29;
t804 = t4.*t9.*t71.*6.800564119502148e-6;
t817 = t2.*t4.*t5.*t71.*1.22799597575967e-5;
t818 = t4.*t5.*t7.*t30.*t72.*4.774692471202153e-30;
t821 = t4.*t7.*t9.*t30.*t72.*4.774692471202153e-30;
t824 = t4.*t6.*t9.*t71.*1.22799597575967e-5;
t825 = t5.*t6.*t8.*t71.*1.22799597575967e-5;
t834 = t5.*t8.*t71.*(-6.800564119502148e-6);
t837 = t4.*t71.*5.537781821510491e-7;
t843 = t2.*t4.*t5.*t71.*1.618032907912407e-6;
t847 = t2.*t8.*t9.*t71.*1.618032907912407e-6;
t848 = t4.*t6.*t9.*t71.*1.618032907912407e-6;
t853 = t2.*t4.*t9.*t71.*6.674437170347525e-6;
t854 = t4.*t5.*t6.*t71.*6.674437170347525e-6;
t855 = t6.*t8.*t9.*t71.*6.674437170347525e-6;
t867 = t4.*t5.*t71.*3.696261130697717e-6;
t870 = t2.*t8.*t71.*2.349236299369594e-6;
t871 = t4.*t6.*t71.*2.349236299369594e-6;
t894 = t8.*t9.*t71.*(-3.696261130697717e-6);
t899 = t2.*t4.*t71.*9.690674399615435e-6;
t902 = t6.*t8.*t71.*9.690674399615435e-6;
t910 = t8.*t71.*5.366634249353632e-6;
t915 = t7.*t17.*t30.*t72.*8.273795699471084e-23;
t917 = t4.*t8.*t30.*t72.*1.391651334125335e-22;
t923 = t4.*t5.*t71.*7.137559230037459e-13;
t924 = t4.*t9.*t71.*7.137559230037459e-13;
t930 = t8.*t71.*7.123247487490083e-7;
t941 = t2.*t4.*t71.*3.021822113324163e-6;
t942 = t6.*t8.*t71.*3.021822113324163e-6;
t943 = t2.*t8.*t71.*1.246511225866906e-5;
t944 = t4.*t6.*t71.*1.246511225866906e-5;
t948 = t4.*t71.*6.903100404659751e-6;
t965 = t7.*t9.*t30.*t72.*9.063852440050829e-23;
t970 = t3.*t30.*t72.*1.268788366711598e-25;
t971 = t16.*t30.*t72.*1.458099973297124e-22;
t972 = t2.*t3.*t9.*t30.*t72.*3.84506501891928e-22;
t973 = t2.*t5.*t7.*t30.*t72.*3.84506501891928e-22;
t974 = t5.*t7.*t30.*t72.*4.926409762458377e-23;
t975 = t6.*t7.*t9.*t30.*t72.*3.84506501891928e-22;
t976 = t2.*t7.*t30.*t72.*5.382450561195517e-25;
t977 = t3.*t6.*t30.*t72.*5.382450561195517e-25;
t978 = t3.*t5.*t8.*t30.*t72.*9.063852440050829e-23;
t979 = t2.*t7.*t9.*t30.*t72.*1.586101540900623e-21;
t980 = t3.*t6.*t9.*t30.*t72.*1.586101540900623e-21;
t981 = t5.*t6.*t7.*t30.*t72.*1.586101540900623e-21;
t984 = t3.*t4.*t30.*t72.*1.313343246602064e-21;
t985 = t3.*t9.*t30.*t72.*1.313343246602064e-21;
t986 = t5.*t7.*t30.*t72.*1.313343246602064e-21;
t989 = t2.*t3.*t4.*t5.*t30.*t72.*3.84506501891928e-22;
t990 = t2.*t3.*t5.*t30.*t72.*2.089880210625419e-22;
t996 = t3.*t5.*t6.*t8.*t30.*t72.*3.84506501891928e-22;
t997 = t2.*t7.*t9.*t30.*t72.*2.089880210625419e-22;
t998 = t5.*t6.*t7.*t30.*t72.*2.089880210625419e-22;
t999 = t3.*t8.*t9.*t30.*t72.*4.926409762458377e-23;
t1002 = t2.*t3.*t30.*t72.*2.220277963292577e-24;
t1003 = t6.*t7.*t30.*t72.*2.220277963292577e-24;
t1004 = t7.*t9.*t30.*t72.*7.138318981153782e-22;
t1007 = t2.*t3.*t8.*t9.*t30.*t72.*(-3.84506501891928e-22);
t1008 = t2.*t5.*t7.*t8.*t30.*t72.*(-3.84506501891928e-22);
t1012 = t2.*t5.*t7.*t30.*t72.*8.620822290548326e-22;
t1013 = t3.*t5.*t6.*t30.*t72.*8.620822290548326e-22;
t1014 = t6.*t7.*t9.*t30.*t72.*8.620822290548326e-22;
t1016 = t3.*t8.*t30.*t72.*9.32742268839803e-25;
t1019 = t30.*t72.*1.170412585872218e-29;
t1020 = t3.*t7.*t30.*t72.*1.650830280755386e-25;
t1021 = t3.*t4.*t30.*t72.*7.138318981153782e-22;
t1022 = t3.*t5.*t30.*t72.*7.138318981153782e-22;
t1023 = t2.*t3.*t5.*t8.*t30.*t72.*1.586101540900623e-21;
t1024 = t3.*t4.*t5.*t6.*t30.*t72.*1.586101540900623e-21;
t1026 = t6.*t30.*t72.*4.965121091065431e-29;
t1027 = t2.*t3.*t4.*t9.*t30.*t72.*2.089880210625419e-22;
t1030 = t3.*t6.*t8.*t9.*t30.*t72.*(-1.586101540900623e-21);
t1031 = t5.*t6.*t7.*t8.*t30.*t72.*(-1.586101540900623e-21);
t1032 = t3.*t8.*t30.*t72.*7.152697935215594e-23;
t1034 = t3.*t6.*t8.*t9.*t30.*t72.*2.089880210625419e-22;
t1035 = t3.*t4.*t7.*t30.*t72.*1.715438754464886e-24;
t1038 = t3.*t8.*t9.*t30.*t72.*(-1.313343246602064e-21);
t1039 = t5.*t7.*t8.*t30.*t72.*(-1.313343246602064e-21);
t1041 = t7.*t30.*t72.*1.150293599235621e-22;
t1043 = t3.*t30.*t72.*1.298466651472986e-21;
t1044 = t2.*t7.*t30.*t72.*2.01292161617043e-21;
t1045 = t3.*t6.*t30.*t72.*2.01292161617043e-21;
t1046 = t2.*t7.*t8.*t9.*t30.*t72.*(-2.089880210625419e-22);
t1048 = t2.*t3.*t8.*t9.*t30.*t72.*8.620822290548326e-22;
t1049 = t3.*t4.*t6.*t9.*t30.*t72.*8.620822290548326e-22;
t1051 = t2.*t3.*t4.*t30.*t72.*3.034315574254804e-22;
t1053 = t2.*t3.*t30.*t72.*4.879772380631159e-22;
t1054 = t2.*t7.*t8.*t30.*t72.*3.034315574254804e-22;
t1055 = t3.*t6.*t8.*t30.*t72.*3.034315574254804e-22;
t1056 = t6.*t7.*t30.*t72.*4.879772380631159e-22;
t1059 = t2.*t30.*t72.*2.048128230484517e-28;
t1061 = t6.*t7.*t8.*t9.*t30.*t72.*(-8.620822290548326e-22);
t1065 = t7.*t8.*t9.*t30.*t72.*(-7.138318981153782e-22);
t1066 = t2.*t3.*t8.*t30.*t72.*1.251664818208198e-21;
t1067 = t3.*t4.*t6.*t30.*t72.*1.251664818208198e-21;
t1068 = t6.*t7.*t8.*t30.*t72.*1.251664818208198e-21;
t1069 = t3.*t4.*t30.*t72.*1.036418850630278e-21;
t1070 = t7.*t8.*t30.*t72.*1.036418850630278e-21;
t1071 = t71.*1.130782628318448e-5;
t1074 = t7.*t30.*t72.*4.303986245035329e-23;
t1075 = t6.*t71.*4.797002992829487e-5;
t1076 = t5.*t7.*t30.*t72.*1.378424649377201e-28;
t1077 = t7.*t9.*t30.*t72.*1.378424649377201e-28;
t1080 = t2.*t71.*1.978778980640035e-4;
t1082 = t3.*t5.*t8.*t30.*t72.*1.378424649377201e-28;
t1083 = t3.*t8.*t9.*t30.*t72.*1.378424649377201e-28;
t1088 = t3.*t4.*t30.*t72.*9.200513714334576e-23;
t1092 = t2.*t3.*t8.*t30.*t72.*3.903039427556764e-22;
t1093 = t2.*t4.*t7.*t30.*t72.*3.903039427556764e-22;
t1094 = t3.*t4.*t6.*t30.*t72.*3.903039427556764e-22;
t1095 = t2.*t3.*t4.*t30.*t72.*1.610016168721029e-21;
t1096 = t3.*t6.*t8.*t30.*t72.*1.610016168721029e-21;
t1097 = t4.*t6.*t7.*t30.*t72.*1.610016168721029e-21;
t1099 = t3.*t8.*t30.*t72.*1.333145329970004e-21;
t1100 = t4.*t7.*t30.*t72.*1.333145329970004e-21;
t1103 = t8.*t9.*t30.*t71.*t72.*9.098517085411002e-23;
t1104 = t4.*t30.*t71.*t72.*1.995717340642186e-24;
t1108 = t8.*t18.*t30.*t71.*t72.*2.829693476925513e-22;
t1109 = t5.*t8.*t9.*t30.*t71.*t72.*1.859969757595868e-22;
t1110 = t5.*t8.*t30.*t71.*t72.*4.945250784909262e-23;
t1117 = t8.*t30.*t71.*t72.*1.41198189047744e-22;
t1118 = t8.*t9.*t16.*t30.*t71.*t72.*1.8197034170822e-22;
t1119 = t16.*t30.*t71.*t72.*3.841105500485731e-25;
t1120 = t4.*t16.*t30.*t71.*t72.*3.991434681284372e-24;
t1123 = t4.*t5.*t30.*t71.*t72.*3.570477686932346e-29;
t1125 = t8.*t16.*t18.*t30.*t71.*t72.*5.659386953851025e-22;
t1127 = t2.*t7.*t30.*t72.*2.750619948951613e-25;
t1130 = t3.*t30.*t72.*3.977152348965926e-22;
t1132 = t5.*t8.*t16.*t30.*t71.*t72.*9.890501569818525e-23;
t1137 = t6.*t7.*t30.*t72.*1.134639471113644e-24;
t1139 = t5.*t8.*t9.*t16.*t30.*t71.*t72.*3.719939515191737e-22;
t1146 = t7.*t30.*t72.*2.158461812807145e-25;
t1149 = t4.*t9.*t30.*t71.*t72.*4.682223280699094e-29;
t1152 = t8.*t16.*t30.*t71.*t72.*2.82396378095488e-22;
t1162 = t4.*t5.*t16.*t30.*t71.*t72.*7.140955373864693e-29;
t1168 = t3.*t30.*t72.*3.979383867109492e-22;
t1180 = t4.*t9.*t16.*t30.*t71.*t72.*9.364446561398189e-29;
t1196 = t30.*t72.*8.661231089831981e-21;
t1206 = t82+t109+t131+t230;
t1207 = t84+t110+t142+t231;
t1219 = t86+t92+t95+t100+t208;
t1270 = t94+t111+t118+t126+t137+t226+t280;
t1271 = t91+t105+t122+t127+t139+t223+t297;
t1272 = t101+t112+t145+t153+t155+t237+t240;
t50 = t27+t28;
t77 = t75.*(3.0./5.0e+2);
t79 = t4.*t5.*t74.*(3.0./5.0e+2);
t80 = t4.*t9.*t74.*(3.0./5.0e+2);
t185 = t75.*8.112963841460668e+31;
t187 = t22.*t76.*3.563742084504373e+31;
t188 = t23.*t76.*3.563742084504373e+31;
t190 = t8.*t75.*3.06620924912759e-3;
t191 = t75.*8.01825475553694e-7;
t198 = t75.*4.35810366141993e-7;
t199 = t5.*t75.*1.603650951107388e-6;
t212 = t18.*t75.*1.639136489385872e-6;
t213 = t52.*t75;
t214 = t9.*t75.*8.71620732283986e-7;
t215 = t8.*t9.*t74.*8.01825475553694e-7;
t220 = t5.*t9.*t75.*2.493725402181286e-6;
t225 = t4.*t74.*1.758766830582798e-8;
t227 = t4.*t5.*t74.*8.01825475553694e-7;
t228 = t4.*t9.*t75.*(-8.01825475553694e-7);
t235 = t5.*t8.*t9.*t74.*1.639136489385872e-6;
t236 = t4.*t5.*t9.*t75.*1.639136489385872e-6;
t238 = t8.*t18.*t74.*2.493725402181286e-6;
t239 = t4.*t18.*t75.*2.493725402181286e-6;
t241 = t4.*t9.*t74.*4.35810366141993e-7;
t242 = t5.*t8.*t74.*4.35810366141993e-7;
t244 = t4.*t5.*t8.*t74.*1.603650951107388e-6;
t245 = t9.*t74.*3.146556677756745e-13;
t256 = t4.*t5.*t8.*t9.*t74.*2.493725402181286e-6;
t263 = t8.*t74.*1.244337995057065e-6;
t264 = t4.*t75.*1.244337995057065e-6;
t265 = t4.*t8.*t18.*t74.*1.639136489385872e-6;
t266 = t4.*t8.*t9.*t74.*8.71620732283986e-7;
t274 = t75.*4.665574824623396e-6;
t283 = t5.*t74.*4.126305279697715e-13;
t284 = t4.*t59.*t74;
t285 = t8.*t59.*t75;
t293 = t9.*t17.*t74.*6.293113355513489e-13;
t300 = t4.*t8.*t74.*5.902365793397849e-7;
t301 = t4.*t5.*t74.*(-3.146556677756745e-13);
t304 = t5.*t8.*t75.*(-3.146556677756745e-13);
t310 = t4.*t62.*t74;
t313 = t9.*t61.*t75;
t323 = t5.*t17.*t74.*8.252610559395431e-13;
t330 = t8.*t74.*8.769009823985418e+48;
t333 = t4.*t5.*t74.*8.4155913e-14;
t334 = t4.*t9.*t74.*8.4155913e-14;
t358 = t17.*t74.*1.458290424491263e-6;
t367 = t183+5.994209437267293e+31;
t380 = t7.*t74.*2.569961002476882e-6;
t385 = t75.*t102;
t416 = -t403;
t475 = t7.*t30.*t47.*t72;
t536 = -t528;
t537 = -t529;
t555 = -t549;
t559 = -t552;
t564 = t74.*8.76226105503051e-2;
t566 = -t561;
t567 = -t563;
t568 = t2.*t4.*t75.*1.324388487819695e-2;
t569 = -t565;
t570 = t4.*t6.*t75.*5.463144604697158e-2;
t572 = t4.*t75.*8.76226105503051e-2;
t574 = t8.*t75.*8.76226105503051e-2;
t575 = t5.*t562;
t576 = t9.*t562;
t577 = t5.*t73.*4.188040994443703e-7;
t578 = t5.*t74.*(-8.76226105503051e-2);
t579 = t75.*1.16331319921549e-5;
t582 = t9.*t73.*2.276295446893622e-7;
t583 = t2.*t74.*4.848080468348049e-9;
t584 = t18.*t73.*2.067207872893371e-6;
t585 = t5.*t9.*t73.*3.144978357570919e-6;
t586 = t74.*1.504998469620115e-8;
t587 = t73.*t253;
t589 = t73.*t246;
t590 = t73.*t247;
t591 = t6.*t74.*1.999848601628674e-8;
t592 = t5.*t16.*t73.*2.022455050551758e-6;
t594 = t3.*t8.*t73.*(-1.545129867076994e-8);
t595 = t75.*1.169554785545351e-5;
t597 = t73.*t276;
t598 = t73.*t277;
t599 = t73.*t278;
t601 = t73.*t282;
t602 = t73.*t271;
t604 = t73.*t272;
t605 = t3.*t4.*t7.*t73.*4.436160944872465e-8;
t606 = t3.*t4.*t18.*t73.*(-2.190813206274814e-6);
t607 = t3.*t4.*t5.*t73.*(-3.828725908394669e-7);
t608 = t16.*t18.*t73.*4.134415745786742e-6;
t609 = t73.*t303;
t610 = t5.*t9.*t16.*t73.*6.289956715141839e-6;
t611 = t3.*t7.*t8.*t9.*t73.*2.022455050551758e-6;
t612 = t73.*t290;
t613 = t3.*t7.*t73.*4.269082063722138e-9;
t615 = t73.*t309;
t616 = t73.*t311;
t618 = t9.*t16.*t73.*1.099250276973348e-6;
t619 = t7.*t9.*t73.*(-2.764345231392299e-13);
t621 = t73.*t306;
t623 = -t614;
t624 = t73.*t308;
t625 = t73.*t320;
t627 = t3.*t5.*t7.*t8.*t9.*t73.*4.134415745786742e-6;
t628 = t3.*t7.*t8.*t18.*t73.*6.289956715141839e-6;
t630 = t73.*t328;
t631 = t73.*t329;
t632 = t73.*t332;
t634 = t3.*t5.*t7.*t8.*t73.*1.099250276973348e-6;
t635 = t4.*t8.*t9.*t73.*(-3.006136635626675e-13);
t636 = t17.*t73.*(-2.81948171692439e-7);
t637 = t5.*t7.*t73.*(-3.625084017661248e-13);
t638 = t3.*t7.*t8.*t73.*3.138610257997577e-6;
t640 = t73.*t338;
t643 = t3.*t4.*t5.*t7.*t73.*7.936601715456896e-13;
t644 = t73.*t345;
t645 = t73.*t346;
t646 = (t3.*t30.*t47.*t72)./8.112963841460668e+31;
t649 = t73.*t348;
t651 = t3.*t8.*t9.*t73.*(-3.625084017661248e-13);
t652 = t4.*t7.*t8.*t73.*(-5.185406908527248e-7);
t654 = t16.*t73.*5.00036577347567e-6;
t656 = t510.*(-1.232595164407831e-32);
t657 = t4.*t5.*t8.*t73.*(-3.94216241479634e-13);
t658 = t73.*t352;
t659 = t4.*t8.*t9.*t16.*t73.*7.936601715456896e-13;
t660 = t510./8.112963841460668e+31;
t661 = t16.*t17.*t73.*7.443807831634578e-7;
t664 = t3.*t4.*t7.*t9.*t73.*1.040783463169498e-12;
t665 = t4.*t5.*t8.*t16.*t73.*1.040783463169498e-12;
t669 = -t666;
t673 = t4.*t8.*t73.*6.966059600064303e-7;
t675 = t73.*t365;
t677 = t5.*t666;
t678 = t9.*t666;
t680 = t7.*t17.*t73.*(-1.281152254279884e-6);
t683 = t5.*t676;
t684 = t9.*t676;
t690 = t4.*t9.*t671;
t698 = t17.*t679;
t699 = t4.*t8.*t16.*t73.*1.83913265673368e-6;
t702 = -t691;
t703 = -t692;
t704 = -t694;
t706 = -t697;
t716 = -t705;
t718 = -t708;
t719 = -t709;
t721 = t4.*t5.*t685;
t725 = -t713;
t728 = -t720;
t730 = -t722;
t731 = -t724;
t734 = -t726;
t737 = t17.*t689;
t739 = -t727;
t740 = t5.*t720;
t741 = -t729;
t742 = t369+2.61156643317655e-1;
t743 = t370+7.38843356682345e-1;
t745 = -t732;
t746 = -t733;
t747 = -t735;
t751 = -t738;
t756 = t9.*t74.*4.172084882644007e-7;
t757 = t372-4.392651260556773e-1;
t759 = -t749;
t762 = t2.*t9.*t75.*1.769880715106441e-6;
t763 = t6.*t9.*t74.*1.769880715106441e-6;
t765 = t9.*t752;
t767 = t2.*t5.*t74.*1.769880715106441e-6;
t770 = t5.*t8.*t75.*4.172084882644007e-7;
t771 = -t764;
t774 = t5.*t74.*2.267622937553823e-7;
t775 = t75.*5.84022389932283e-10;
t777 = t75.*t390;
t778 = t2.*t9.*t74.*7.30081420113316e-6;
t779 = t5.*t6.*t74.*7.30081420113316e-6;
t781 = t6.*t9.*t75.*7.30081420113316e-6;
t787 = -t773;
t788 = t2.*t74.*2.477538195427268e-9;
t790 = t6.*t75.*2.477538195427268e-9;
t795 = t75.*t388;
t796 = t2.*t8.*t9.*t75.*(-1.769880715106441e-6);
t797 = t5.*t6.*t8.*t75.*(-1.769880715106441e-6);
t801 = -t782;
t802 = -t783;
t803 = -t784;
t805 = t5.*t773;
t810 = -t786;
t811 = t3.*t9.*t73.*6.735277470591094e-6;
t812 = t2.*t75.*1.021992379861453e-8;
t813 = t6.*t74.*1.021992379861453e-8;
t814 = t5.*t74.*1.170967356229242e-5;
t816 = t4.*t75.*1.170967356229242e-5;
t819 = t9.*t75.*1.170967356229242e-5;
t820 = t4.*t5.*t73.*1.132872773043163e-5;
t822 = -t792;
t823 = t8.*t9.*t75.*2.267622937553823e-7;
t826 = -t798;
t828 = -t799;
t829 = t2.*t9.*t74.*9.619703863182361e-7;
t830 = t2.*t5.*t75.*9.619703863182361e-7;
t831 = t5.*t6.*t74.*9.619703863182361e-7;
t833 = -t804;
t836 = t74.*5.29479332073745e-7;
t838 = t2.*t5.*t74.*3.96815841743287e-6;
t839 = -t818;
t841 = t6.*t9.*t74.*3.96815841743287e-6;
t842 = t5.*t6.*t75.*3.96815841743287e-6;
t844 = t3.*t5.*t73.*3.660776353481749e-6;
t845 = -t824;
t846 = -t825;
t849 = t75.*t406;
t851 = t75.*t407;
t852 = t6.*t8.*t9.*t75.*(-7.30081420113316e-6);
t856 = t5.*t7.*t8.*t73.*6.735277470591094e-6;
t859 = t4.*t75.*6.364473664374288e-6;
t860 = t9.*t74.*6.364473664374288e-6;
t861 = t5.*t75.*6.364473664374288e-6;
t862 = t8.*t75.*3.292381812591008e-7;
t869 = t4.*t9.*t73.*6.157420948384101e-6;
t872 = t9.*t798;
t873 = -t847;
t874 = -t848;
t876 = t75.*t446;
t878 = t75.*t428;
t879 = -t855;
t880 = t2.*t8.*t74.*1.396693317797299e-6;
t881 = t75.*t429;
t883 = t75.*t430;
t884 = t2.*t75.*2.246155783606385e-6;
t885 = t6.*t74.*2.246155783606385e-6;
t886 = t8.*t9.*t75.*(-1.170967356229242e-5);
t887 = t75.*t432;
t889 = t75.*t433;
t891 = t7.*t8.*t9.*t73.*3.660776353481749e-6;
t892 = -t870;
t893 = -t871;
t895 = t75.*t466;
t896 = t6.*t8.*t74.*5.761404326386517e-6;
t897 = t75.*t467;
t898 = t3.*t73.*2.844856587289647e-6;
t900 = t6.*t8.*t9.*t75.*(-9.619703863182361e-7);
t901 = t4.*t73.*8.940013971103833e-6;
t906 = t75.*8.369355329119605e-6;
t907 = t6.*t8.*t75.*(-1.396693317797299e-6);
t908 = t2.*t74.*9.26546399593074e-6;
t909 = t6.*t75.*9.26546399593074e-6;
t912 = -t902;
t914 = -t910;
t916 = t7.*t8.*t73.*5.315113587256377e-6;
t918 = t8.*t74.*9.240635641966378e-6;
t919 = t4.*t75.*9.240635641966378e-6;
t920 = t74.*7.425831767740348e-7;
t921 = t7.*t73.*6.474095421643823e-7;
t922 = -t917;
t925 = t5.*t74.*1.228993465050726e-12;
t926 = t9.*t74.*1.228993465050726e-12;
t927 = -t923;
t928 = -t924;
t931 = t5.*t8.*t75.*1.228993465050726e-12;
t932 = t8.*t9.*t75.*1.228993465050726e-12;
t933 = t4.*t75.*4.23498997076776e-7;
t938 = t2.*t4.*t74.*1.796566294495167e-6;
t939 = t75.*t534;
t940 = t75.*t535;
t945 = t8.*t73.*1.14995379215611e-5;
t946 = t75+t527;
t949 = -t942;
t951 = t75.*t539;
t952 = t4.*t6.*t74.*7.410893064247368e-6;
t954 = t75.*t540;
t955 = t4.*t74.*1.188622750787503e-5;
t956 = t8.*t75.*1.188622750787503e-5;
t957 = t2.*t4.*t75.*(-7.410893064247368e-6);
t960 = t4.*t7.*t73.*6.836829388815e-6;
t968 = -t965;
t982 = -t972;
t983 = -t973;
t987 = -t976;
t988 = -t977;
t991 = -t979;
t992 = -t980;
t993 = -t981;
t994 = t8.*t972;
H = ft_2({t1002,t1003,t1004,t1007,t1008,t101,t1012,t1013,t1014,t1016,t1019,t102,t1020,t1021,t1022,t1023,t1024,t1026,t1027,t1030,t1031,t1032,t1034,t1035,t1038,t1039,t1041,t1043,t1044,t1045,t1046,t1048,t1049,t1051,t1053,t1054,t1055,t1056,t1059,t106,t1061,t1065,t1066,t1067,t1068,t1069,t107,t1070,t1071,t1074,t1075,t1076,t1077,t108,t1080,t1082,t1083,t1088,t1090,t1092,t1093,t1094,t1095,t1096,t1097,t1099,t1100,t1103,t1104,t1108,t1109,t1110,t1117,t1118,t1119,t1120,t1123,t1125,t1127,t113,t1130,t1132,t1137,t1139,t114,t1146,t1149,t115,t1152,t1162,t1168,t1180,t119,t1196,t120,t1206,t1207,t121,t1219,t124,t1270,t1271,t1272,t130,t132,t133,t134,t135,t136,t138,t14,t140,t141,t144,t146,t149,t15,t150,t151,t152,t153,t154,t156,t158,t159,t16,t160,t161,t162,t163,t164,t166,t167,t168,t169,t17,t170,t171,t172,t175,t177,t178,t179,t18,t180,t181,t184,t185,t186,t187,t188,t189,t19,t190,t191,t192,t194,t196,t197,t198,t199,t2,t20,t200,t202,t203,t204,t209,t21,t210,t211,t212,t213,t214,t215,t217,t218,t219,t22,t220,t221,t222,t225,t227,t228,t23,t232,t233,t234,t235,t236,t237,t238,t239,t240,t241,t242,t244,t245,t246,t248,t251,t255,t256,t257,t258,t26,t260,t261,t262,t263,t264,t265,t266,t267,t268,t27,t273,t274,t278,t282,t283,t287,t288,t289,t291,t292,t293,t294,t295,t296,t298,t3,t30,t300,t301,t302,t303,t304,t305,t307,t310,t313,t315,t316,t319,t321,t322,t323,t326,t327,t328,t329,t330,t331,t332,t333,t334,t336,t337,t340,t341,t343,t344,t345,t346,t347,t348,t349,t35,t351,t353,t354,t355,t356,t357,t358,t361,t362,t364,t365,t366,t367,t368,t373,t374,t377,t379,t38,t380,t381,t382,t383,t384,t385,t386,t387,t388,t391,t393,t394,t395,t396,t397,t4,t401,t402,t404,t405,t406,t407,t408,t409,t41,t412,t413,t414,t415,t416,t419,t42,t420,t423,t424,t425,t426,t427,t429,t43,t432,t433,t434,t435,t436,t437,t441,t442,t446,t447,t448,t449,t45,t450,t451,t452,t453,t454,t455,t458,t459,t460,t461,t463,t464,t465,t466,t467,t468,t469,t47,t470,t471,t472,t473,t474,t475,t476,t477,t478,t479,t480,t486,t489,t493,t494,t495,t496,t497,t498,t499,t5,t500,t501,t503,t505,t506,t507,t508,t509,t510,t511,t512,t514,t515,t518,t519,t520,t521,t522,t523,t524,t528,t529,t530,t531,t532,t533,t534,t535,t536,t537,t538,t540,t541,t543,t544,t545,t546,t548,t550,t551,t553,t554,t555,t557,t558,t559,t560,t562,t564,t566,t567,t568,t569,t570,t572,t574,t575,t576,t577,t578,t579,t582,t583,t584,t585,t586,t587,t588,t59,t590,t591,t592,t593,t594,t595,t596,t597,t598,t6,t602,t603,t604,t605,t606,t607,t608,t610,t611,t612,t613,t615,t616,t618,t619,t62,t621,t623,t624,t625,t627,t628,t634,t635,t636,t637,t638,t640,t643,t646,t651,t652,t653,t654,t657,t658,t659,t660,t661,t664,t665,t668,t669,t670,t671,t672,t673,t674,t676,t677,t679,t680,t681,t682,t683,t684,t685,t686,t687,t688,t689,t693,t695,t696,t699,t7,t700,t701,t702,t703,t704,t706,t707,t71,t710,t711,t712,t714,t715,t716,t717,t718,t719,t72,t720,t721,t723,t725,t728,t73,t730,t731,t734,t736,t739,t74,t741,t742,t743,t744,t745,t746,t747,t748,t75,t750,t751,t752,t753,t754,t755,t756,t757,t758,t759,t760,t761,t762,t763,t765,t766,t767,t77,t770,t771,t772,t773,t774,t775,t778,t779,t78,t780,t781,t785,t786,t787,t788,t789,t79,t790,t791,t795,t796,t797,t8,t80,t801,t802,t803,t810,t811,t812,t813,t814,t816,t817,t819,t820,t821,t822,t823,t826,t828,t829,t830,t831,t833,t834,t836,t837,t838,t839,t841,t842,t843,t844,t845,t846,t849,t85,t851,t852,t853,t854,t856,t859,t860,t861,t862,t867,t869,t87,t873,t874,t876,t879,t88,t880,t881,t884,t885,t886,t887,t889,t89,t891,t892,t893,t894,t895,t896,t897,t898,t899,t9,t90,t900,t901,t906,t907,t908,t909,t912,t914,t915,t916,t918,t919,t920,t921,t922,t923,t925,t926,t927,t928,t930,t931,t932,t933,t938,t939,t940,t941,t943,t944,t945,t946,t948,t949,t952,t954,t955,t956,t957,t96,t960,t968,t970,t971,t973,t974,t975,t978,t980,t981,t982,t983,t984,t985,t986,t987,t988,t989,t990,t991,t992,t993,t996,t997,t998,t999});
end
function H = ft_2(ct)
t1002 = ct{1};
t1003 = ct{2};
t1004 = ct{3};
t1007 = ct{4};
t1008 = ct{5};
t101 = ct{6};
t1012 = ct{7};
t1013 = ct{8};
t1014 = ct{9};
t1016 = ct{10};
t1019 = ct{11};
t102 = ct{12};
t1020 = ct{13};
t1021 = ct{14};
t1022 = ct{15};
t1023 = ct{16};
t1024 = ct{17};
t1026 = ct{18};
t1027 = ct{19};
t1030 = ct{20};
t1031 = ct{21};
t1032 = ct{22};
t1034 = ct{23};
t1035 = ct{24};
t1038 = ct{25};
t1039 = ct{26};
t1041 = ct{27};
t1043 = ct{28};
t1044 = ct{29};
t1045 = ct{30};
t1046 = ct{31};
t1048 = ct{32};
t1049 = ct{33};
t1051 = ct{34};
t1053 = ct{35};
t1054 = ct{36};
t1055 = ct{37};
t1056 = ct{38};
t1059 = ct{39};
t106 = ct{40};
t1061 = ct{41};
t1065 = ct{42};
t1066 = ct{43};
t1067 = ct{44};
t1068 = ct{45};
t1069 = ct{46};
t107 = ct{47};
t1070 = ct{48};
t1071 = ct{49};
t1074 = ct{50};
t1075 = ct{51};
t1076 = ct{52};
t1077 = ct{53};
t108 = ct{54};
t1080 = ct{55};
t1082 = ct{56};
t1083 = ct{57};
t1088 = ct{58};
t1090 = ct{59};
t1092 = ct{60};
t1093 = ct{61};
t1094 = ct{62};
t1095 = ct{63};
t1096 = ct{64};
t1097 = ct{65};
t1099 = ct{66};
t1100 = ct{67};
t1103 = ct{68};
t1104 = ct{69};
t1108 = ct{70};
t1109 = ct{71};
t1110 = ct{72};
t1117 = ct{73};
t1118 = ct{74};
t1119 = ct{75};
t1120 = ct{76};
t1123 = ct{77};
t1125 = ct{78};
t1127 = ct{79};
t113 = ct{80};
t1130 = ct{81};
t1132 = ct{82};
t1137 = ct{83};
t1139 = ct{84};
t114 = ct{85};
t1146 = ct{86};
t1149 = ct{87};
t115 = ct{88};
t1152 = ct{89};
t1162 = ct{90};
t1168 = ct{91};
t1180 = ct{92};
t119 = ct{93};
t1196 = ct{94};
t120 = ct{95};
t1206 = ct{96};
t1207 = ct{97};
t121 = ct{98};
t1219 = ct{99};
t124 = ct{100};
t1270 = ct{101};
t1271 = ct{102};
t1272 = ct{103};
t130 = ct{104};
t132 = ct{105};
t133 = ct{106};
t134 = ct{107};
t135 = ct{108};
t136 = ct{109};
t138 = ct{110};
t14 = ct{111};
t140 = ct{112};
t141 = ct{113};
t144 = ct{114};
t146 = ct{115};
t149 = ct{116};
t15 = ct{117};
t150 = ct{118};
t151 = ct{119};
t152 = ct{120};
t153 = ct{121};
t154 = ct{122};
t156 = ct{123};
t158 = ct{124};
t159 = ct{125};
t16 = ct{126};
t160 = ct{127};
t161 = ct{128};
t162 = ct{129};
t163 = ct{130};
t164 = ct{131};
t166 = ct{132};
t167 = ct{133};
t168 = ct{134};
t169 = ct{135};
t17 = ct{136};
t170 = ct{137};
t171 = ct{138};
t172 = ct{139};
t175 = ct{140};
t177 = ct{141};
t178 = ct{142};
t179 = ct{143};
t18 = ct{144};
t180 = ct{145};
t181 = ct{146};
t184 = ct{147};
t185 = ct{148};
t186 = ct{149};
t187 = ct{150};
t188 = ct{151};
t189 = ct{152};
t19 = ct{153};
t190 = ct{154};
t191 = ct{155};
t192 = ct{156};
t194 = ct{157};
t196 = ct{158};
t197 = ct{159};
t198 = ct{160};
t199 = ct{161};
t2 = ct{162};
t20 = ct{163};
t200 = ct{164};
t202 = ct{165};
t203 = ct{166};
t204 = ct{167};
t209 = ct{168};
t21 = ct{169};
t210 = ct{170};
t211 = ct{171};
t212 = ct{172};
t213 = ct{173};
t214 = ct{174};
t215 = ct{175};
t217 = ct{176};
t218 = ct{177};
t219 = ct{178};
t22 = ct{179};
t220 = ct{180};
t221 = ct{181};
t222 = ct{182};
t225 = ct{183};
t227 = ct{184};
t228 = ct{185};
t23 = ct{186};
t232 = ct{187};
t233 = ct{188};
t234 = ct{189};
t235 = ct{190};
t236 = ct{191};
t237 = ct{192};
t238 = ct{193};
t239 = ct{194};
t240 = ct{195};
t241 = ct{196};
t242 = ct{197};
t244 = ct{198};
t245 = ct{199};
t246 = ct{200};
t248 = ct{201};
t251 = ct{202};
t255 = ct{203};
t256 = ct{204};
t257 = ct{205};
t258 = ct{206};
t26 = ct{207};
t260 = ct{208};
t261 = ct{209};
t262 = ct{210};
t263 = ct{211};
t264 = ct{212};
t265 = ct{213};
t266 = ct{214};
t267 = ct{215};
t268 = ct{216};
t27 = ct{217};
t273 = ct{218};
t274 = ct{219};
t278 = ct{220};
t282 = ct{221};
t283 = ct{222};
t287 = ct{223};
t288 = ct{224};
t289 = ct{225};
t291 = ct{226};
t292 = ct{227};
t293 = ct{228};
t294 = ct{229};
t295 = ct{230};
t296 = ct{231};
t298 = ct{232};
t3 = ct{233};
t30 = ct{234};
t300 = ct{235};
t301 = ct{236};
t302 = ct{237};
t303 = ct{238};
t304 = ct{239};
t305 = ct{240};
t307 = ct{241};
t310 = ct{242};
t313 = ct{243};
t315 = ct{244};
t316 = ct{245};
t319 = ct{246};
t321 = ct{247};
t322 = ct{248};
t323 = ct{249};
t326 = ct{250};
t327 = ct{251};
t328 = ct{252};
t329 = ct{253};
t330 = ct{254};
t331 = ct{255};
t332 = ct{256};
t333 = ct{257};
t334 = ct{258};
t336 = ct{259};
t337 = ct{260};
t340 = ct{261};
t341 = ct{262};
t343 = ct{263};
t344 = ct{264};
t345 = ct{265};
t346 = ct{266};
t347 = ct{267};
t348 = ct{268};
t349 = ct{269};
t35 = ct{270};
t351 = ct{271};
t353 = ct{272};
t354 = ct{273};
t355 = ct{274};
t356 = ct{275};
t357 = ct{276};
t358 = ct{277};
t361 = ct{278};
t362 = ct{279};
t364 = ct{280};
t365 = ct{281};
t366 = ct{282};
t367 = ct{283};
t368 = ct{284};
t373 = ct{285};
t374 = ct{286};
t377 = ct{287};
t379 = ct{288};
t38 = ct{289};
t380 = ct{290};
t381 = ct{291};
t382 = ct{292};
t383 = ct{293};
t384 = ct{294};
t385 = ct{295};
t386 = ct{296};
t387 = ct{297};
t388 = ct{298};
t391 = ct{299};
t393 = ct{300};
t394 = ct{301};
t395 = ct{302};
t396 = ct{303};
t397 = ct{304};
t4 = ct{305};
t401 = ct{306};
t402 = ct{307};
t404 = ct{308};
t405 = ct{309};
t406 = ct{310};
t407 = ct{311};
t408 = ct{312};
t409 = ct{313};
t41 = ct{314};
t412 = ct{315};
t413 = ct{316};
t414 = ct{317};
t415 = ct{318};
t416 = ct{319};
t419 = ct{320};
t42 = ct{321};
t420 = ct{322};
t423 = ct{323};
t424 = ct{324};
t425 = ct{325};
t426 = ct{326};
t427 = ct{327};
t429 = ct{328};
t43 = ct{329};
t432 = ct{330};
t433 = ct{331};
t434 = ct{332};
t435 = ct{333};
t436 = ct{334};
t437 = ct{335};
t441 = ct{336};
t442 = ct{337};
t446 = ct{338};
t447 = ct{339};
t448 = ct{340};
t449 = ct{341};
t45 = ct{342};
t450 = ct{343};
t451 = ct{344};
t452 = ct{345};
t453 = ct{346};
t454 = ct{347};
t455 = ct{348};
t458 = ct{349};
t459 = ct{350};
t460 = ct{351};
t461 = ct{352};
t463 = ct{353};
t464 = ct{354};
t465 = ct{355};
t466 = ct{356};
t467 = ct{357};
t468 = ct{358};
t469 = ct{359};
t47 = ct{360};
t470 = ct{361};
t471 = ct{362};
t472 = ct{363};
t473 = ct{364};
t474 = ct{365};
t475 = ct{366};
t476 = ct{367};
t477 = ct{368};
t478 = ct{369};
t479 = ct{370};
t480 = ct{371};
t486 = ct{372};
t489 = ct{373};
t493 = ct{374};
t494 = ct{375};
t495 = ct{376};
t496 = ct{377};
t497 = ct{378};
t498 = ct{379};
t499 = ct{380};
t5 = ct{381};
t500 = ct{382};
t501 = ct{383};
t503 = ct{384};
t505 = ct{385};
t506 = ct{386};
t507 = ct{387};
t508 = ct{388};
t509 = ct{389};
t510 = ct{390};
t511 = ct{391};
t512 = ct{392};
t514 = ct{393};
t515 = ct{394};
t518 = ct{395};
t519 = ct{396};
t520 = ct{397};
t521 = ct{398};
t522 = ct{399};
t523 = ct{400};
t524 = ct{401};
t528 = ct{402};
t529 = ct{403};
t530 = ct{404};
t531 = ct{405};
t532 = ct{406};
t533 = ct{407};
t534 = ct{408};
t535 = ct{409};
t536 = ct{410};
t537 = ct{411};
t538 = ct{412};
t540 = ct{413};
t541 = ct{414};
t543 = ct{415};
t544 = ct{416};
t545 = ct{417};
t546 = ct{418};
t548 = ct{419};
t550 = ct{420};
t551 = ct{421};
t553 = ct{422};
t554 = ct{423};
t555 = ct{424};
t557 = ct{425};
t558 = ct{426};
t559 = ct{427};
t560 = ct{428};
t562 = ct{429};
t564 = ct{430};
t566 = ct{431};
t567 = ct{432};
t568 = ct{433};
t569 = ct{434};
t570 = ct{435};
t572 = ct{436};
t574 = ct{437};
t575 = ct{438};
t576 = ct{439};
t577 = ct{440};
t578 = ct{441};
t579 = ct{442};
t582 = ct{443};
t583 = ct{444};
t584 = ct{445};
t585 = ct{446};
t586 = ct{447};
t587 = ct{448};
t588 = ct{449};
t59 = ct{450};
t590 = ct{451};
t591 = ct{452};
t592 = ct{453};
t593 = ct{454};
t594 = ct{455};
t595 = ct{456};
t596 = ct{457};
t597 = ct{458};
t598 = ct{459};
t6 = ct{460};
t602 = ct{461};
t603 = ct{462};
t604 = ct{463};
t605 = ct{464};
t606 = ct{465};
t607 = ct{466};
t608 = ct{467};
t610 = ct{468};
t611 = ct{469};
t612 = ct{470};
t613 = ct{471};
t615 = ct{472};
t616 = ct{473};
t618 = ct{474};
t619 = ct{475};
t62 = ct{476};
t621 = ct{477};
t623 = ct{478};
t624 = ct{479};
t625 = ct{480};
t627 = ct{481};
t628 = ct{482};
t634 = ct{483};
t635 = ct{484};
t636 = ct{485};
t637 = ct{486};
t638 = ct{487};
t640 = ct{488};
t643 = ct{489};
t646 = ct{490};
t651 = ct{491};
t652 = ct{492};
t653 = ct{493};
t654 = ct{494};
t657 = ct{495};
t658 = ct{496};
t659 = ct{497};
t660 = ct{498};
t661 = ct{499};
t664 = ct{500};
t665 = ct{501};
t668 = ct{502};
t669 = ct{503};
t670 = ct{504};
t671 = ct{505};
t672 = ct{506};
t673 = ct{507};
t674 = ct{508};
t676 = ct{509};
t677 = ct{510};
t679 = ct{511};
t680 = ct{512};
t681 = ct{513};
t682 = ct{514};
t683 = ct{515};
t684 = ct{516};
t685 = ct{517};
t686 = ct{518};
t687 = ct{519};
t688 = ct{520};
t689 = ct{521};
t693 = ct{522};
t695 = ct{523};
t696 = ct{524};
t699 = ct{525};
t7 = ct{526};
t700 = ct{527};
t701 = ct{528};
t702 = ct{529};
t703 = ct{530};
t704 = ct{531};
t706 = ct{532};
t707 = ct{533};
t71 = ct{534};
t710 = ct{535};
t711 = ct{536};
t712 = ct{537};
t714 = ct{538};
t715 = ct{539};
t716 = ct{540};
t717 = ct{541};
t718 = ct{542};
t719 = ct{543};
t72 = ct{544};
t720 = ct{545};
t721 = ct{546};
t723 = ct{547};
t725 = ct{548};
t728 = ct{549};
t73 = ct{550};
t730 = ct{551};
t731 = ct{552};
t734 = ct{553};
t736 = ct{554};
t739 = ct{555};
t74 = ct{556};
t741 = ct{557};
t742 = ct{558};
t743 = ct{559};
t744 = ct{560};
t745 = ct{561};
t746 = ct{562};
t747 = ct{563};
t748 = ct{564};
t75 = ct{565};
t750 = ct{566};
t751 = ct{567};
t752 = ct{568};
t753 = ct{569};
t754 = ct{570};
t755 = ct{571};
t756 = ct{572};
t757 = ct{573};
t758 = ct{574};
t759 = ct{575};
t760 = ct{576};
t761 = ct{577};
t762 = ct{578};
t763 = ct{579};
t765 = ct{580};
t766 = ct{581};
t767 = ct{582};
t77 = ct{583};
t770 = ct{584};
t771 = ct{585};
t772 = ct{586};
t773 = ct{587};
t774 = ct{588};
t775 = ct{589};
t778 = ct{590};
t779 = ct{591};
t78 = ct{592};
t780 = ct{593};
t781 = ct{594};
t785 = ct{595};
t786 = ct{596};
t787 = ct{597};
t788 = ct{598};
t789 = ct{599};
t79 = ct{600};
t790 = ct{601};
t791 = ct{602};
t795 = ct{603};
t796 = ct{604};
t797 = ct{605};
t8 = ct{606};
t80 = ct{607};
t801 = ct{608};
t802 = ct{609};
t803 = ct{610};
t810 = ct{611};
t811 = ct{612};
t812 = ct{613};
t813 = ct{614};
t814 = ct{615};
t816 = ct{616};
t817 = ct{617};
t819 = ct{618};
t820 = ct{619};
t821 = ct{620};
t822 = ct{621};
t823 = ct{622};
t826 = ct{623};
t828 = ct{624};
t829 = ct{625};
t830 = ct{626};
t831 = ct{627};
t833 = ct{628};
t834 = ct{629};
t836 = ct{630};
t837 = ct{631};
t838 = ct{632};
t839 = ct{633};
t841 = ct{634};
t842 = ct{635};
t843 = ct{636};
t844 = ct{637};
t845 = ct{638};
t846 = ct{639};
t849 = ct{640};
t85 = ct{641};
t851 = ct{642};
t852 = ct{643};
t853 = ct{644};
t854 = ct{645};
t856 = ct{646};
t859 = ct{647};
t860 = ct{648};
t861 = ct{649};
t862 = ct{650};
t867 = ct{651};
t869 = ct{652};
t87 = ct{653};
t873 = ct{654};
t874 = ct{655};
t876 = ct{656};
t879 = ct{657};
t88 = ct{658};
t880 = ct{659};
t881 = ct{660};
t884 = ct{661};
t885 = ct{662};
t886 = ct{663};
t887 = ct{664};
t889 = ct{665};
t89 = ct{666};
t891 = ct{667};
t892 = ct{668};
t893 = ct{669};
t894 = ct{670};
t895 = ct{671};
t896 = ct{672};
t897 = ct{673};
t898 = ct{674};
t899 = ct{675};
t9 = ct{676};
t90 = ct{677};
t900 = ct{678};
t901 = ct{679};
t906 = ct{680};
t907 = ct{681};
t908 = ct{682};
t909 = ct{683};
t912 = ct{684};
t914 = ct{685};
t915 = ct{686};
t916 = ct{687};
t918 = ct{688};
t919 = ct{689};
t920 = ct{690};
t921 = ct{691};
t922 = ct{692};
t923 = ct{693};
t925 = ct{694};
t926 = ct{695};
t927 = ct{696};
t928 = ct{697};
t930 = ct{698};
t931 = ct{699};
t932 = ct{700};
t933 = ct{701};
t938 = ct{702};
t939 = ct{703};
t940 = ct{704};
t941 = ct{705};
t943 = ct{706};
t944 = ct{707};
t945 = ct{708};
t946 = ct{709};
t948 = ct{710};
t949 = ct{711};
t952 = ct{712};
t954 = ct{713};
t955 = ct{714};
t956 = ct{715};
t957 = ct{716};
t96 = ct{717};
t960 = ct{718};
t968 = ct{719};
t970 = ct{720};
t971 = ct{721};
t973 = ct{722};
t974 = ct{723};
t975 = ct{724};
t978 = ct{725};
t980 = ct{726};
t981 = ct{727};
t982 = ct{728};
t983 = ct{729};
t984 = ct{730};
t985 = ct{731};
t986 = ct{732};
t987 = ct{733};
t988 = ct{734};
t989 = ct{735};
t990 = ct{736};
t991 = ct{737};
t992 = ct{738};
t993 = ct{739};
t996 = ct{740};
t997 = ct{741};
t998 = ct{742};
t999 = ct{743};
t995 = t8.*t973;
t1000 = -t985;
t1001 = -t986;
t1005 = t8.*t980;
t1006 = t8.*t981;
t1009 = -t996;
t1010 = -t997;
t1011 = -t998;
t1015 = t5.*t984;
t1017 = t8.*t985;
t1018 = t8.*t986;
t1025 = -t1003;
t1028 = t8.*t990;
t1029 = -t1004;
t1033 = t8.*t997;
t1036 = -t1014;
t1037 = -t1016;
t1040 = -t1020;
t1042 = -t1026;
t1047 = -t1034;
t1050 = t8.*t1013;
t1052 = t8.*t1014;
t1057 = t9.*t1021;
t1058 = t8.*t1022;
t1060 = t8.*t1004;
t1062 = -t1054;
t1063 = -t1055;
t1064 = -t1056;
t1072 = -t1068;
t1073 = -t1070;
t1078 = -t1074;
t1079 = -t1075;
t1081 = -t1076;
t1085 = -t1082;
t1086 = -t1083;
t1089 = -t1088;
t1101 = -t1095;
t1102 = t73.*7.67777073541389e-5;
t1105 = -t1103;
t1106 = -t1104;
t1107 = t5.*t7.*t30.*t72.*t74.*1.8197034170822e-22;
t1111 = t4.*t9.*t30.*t72.*t75.*1.530369361342075e-22;
t1112 = t5.*t7.*t9.*t30.*t72.*t74.*5.659386953851025e-22;
t1113 = t8.*t30.*t72.*t75.*3.356793907564468e-24;
t1114 = -t1109;
t1115 = t7.*t18.*t30.*t72.*t74.*3.719939515191737e-22;
t1121 = t7.*t9.*t30.*t72.*t74.*9.890501569818525e-23;
t1122 = t4.*t5.*t9.*t30.*t72.*t75.*3.128466653771177e-22;
t1124 = -t1117;
t1126 = -t1119;
t1128 = t4.*t5.*t8.*t30.*t72.*t74.*3.060738722684151e-22;
t1129 = t4.*t18.*t30.*t72.*t75.*4.759540657477059e-22;
t1134 = -t1125;
t1135 = t9.*t30.*t72.*t74.*6.005538711575609e-29;
t1136 = t4.*t5.*t30.*t72.*t75.*8.317905230417136e-23;
t1138 = -t1127;
t1140 = -t1132;
t1141 = t5.*t7.*t17.*t30.*t72.*t74.*(-1.8197034170822e-22);
t1142 = t4.*t5.*t8.*t9.*t30.*t72.*t74.*4.759540657477059e-22;
t1143 = t4.*t8.*t18.*t30.*t72.*t74.*3.128466653771177e-22;
t1144 = t4.*t8.*t9.*t30.*t72.*t74.*1.663581046083427e-22;
t1147 = -t1137;
t1148 = t4.*t30.*t72.*t75.*2.374951658244784e-22;
t1150 = t7.*t17.*t18.*t30.*t72.*t74.*1.859969757595868e-22;
t1151 = t5.*t8.*t30.*t72.*t75.*6.005538711575609e-29;
t1153 = t5.*t7.*t9.*t17.*t30.*t72.*t74.*2.829693476925513e-22;
t1154 = -t1146;
t1157 = t5.*t30.*t72.*t74.*7.875493318833269e-29;
t1158 = -t1149;
t1163 = t7.*t30.*t72.*t74.*4.499077832247571e-22;
t1169 = t7.*t9.*t17.*t30.*t72.*t74.*(-9.890501569818525e-23);
t1171 = t4.*t8.*t30.*t72.*t74.*1.126529406341455e-22;
t1172 = -t1162;
t1175 = t9.*t17.*t30.*t72.*t74.*1.201107742315122e-28;
t1176 = t8.*t9.*t30.*t72.*t75.*7.875493318833269e-29;
t1178 = t4.*t7.*t8.*t9.*t30.*t72.*t74.*7.140955373864693e-29;
t1179 = t5.*t17.*t30.*t72.*t74.*1.575098663766654e-28;
t1181 = t7.*t17.*t30.*t72.*t74.*6.697564202296239e-23;
t1183 = t4.*t5.*t7.*t8.*t30.*t72.*t74.*9.364446561398189e-29;
t1189 = t17.*t30.*t72.*t74.*2.783302668250669e-22;
t1191 = t4.*t7.*t8.*t30.*t72.*t74.*1.654759139894217e-22;
t1193 = t9.*t30.*t72.*t75.*1.463238712860231e-21;
t1195 = t5.*t30.*t72.*t75.*7.953034901571333e-22;
t1197 = t5.*t8.*t30.*t72.*t74.*1.463238712860231e-21;
t1198 = -t1196;
t1199 = t8.*t9.*t30.*t72.*t74.*7.953034901571333e-22;
t1200 = t30.*t72.*t75.*6.180449594294637e-22;
t1201 = t8.*t30.*t72.*t74.*1.154708176178584e-21;
t1202 = t30.*t72.*t74.*1.406496925043394e-22;
t1203 = t4.*t30.*t72.*t74.*1.485300862305337e-21;
t81 = -t79;
t216 = t4.*t9.*t191;
t243 = t4.*t5.*t198;
t250 = -t236;
t252 = -t238;
t254 = -t242;
t259 = -t245;
t279 = -t264;
t299 = -t283;
t314 = -t300;
t339 = -t330;
t342 = -t334;
t359 = -t358;
t375 = t22.*t367;
t376 = t23.*t367;
t504 = -t475;
t571 = t5.*t564;
t573 = t9.*t564;
t580 = t5.*t574;
t581 = t9.*t574;
t600 = -t592;
t617 = -t608;
t620 = -t610;
t622 = -t613;
t626 = t17.*t592;
t629 = -t618;
t633 = -t628;
t639 = t16.*t17.*t584;
t641 = t16.*t17.*t585;
t642 = -t634;
t647 = t475./8.112963841460668e+31;
t648 = t17.*t618;
t650 = -t643;
t662 = -t659;
t663 = -t661;
t667 = -t665;
t768 = -t762;
t769 = -t763;
t776 = t8.*t762;
t793 = -t774;
t794 = t8.*t767;
t800 = -t781;
t806 = t22.*t742;
t807 = t22.*t743;
t808 = t23.*t742;
t809 = t23.*t743;
t815 = -t790;
t827 = t8.*t781;
t832 = t22.*t757;
t835 = t23.*t757;
t840 = -t819;
t850 = t8.*t779;
t858 = -t836;
t863 = t8.*t814;
t864 = t5.*t816;
t865 = t8.*t819;
t866 = -t838;
t868 = -t844;
t875 = t8.*t829;
t877 = t8.*t830;
t888 = t8.*t841;
t890 = t8.*t842;
t903 = t8.*t860;
t904 = t9.*t859;
t905 = t8.*t861;
t911 = -t898;
t913 = -t908;
t929 = -t926;
t934 = -t931;
t935 = -t932;
t936 = -t933;
t937 = t185+t340;
t947 = -t938;
t950 = t74+t536;
t958 = -t952;
t959 = t946.^2;
t961 = -t955;
t962 = t5.*t946;
t963 = t9.*t946;
t964 = -t960;
t1116 = -t1111;
t1131 = -t1122;
t1133 = t17.*t1107;
t1145 = -t1135;
t1155 = -t1148;
t1156 = t17.*t1121;
t1159 = -t1150;
t1160 = -t1151;
t1161 = t41.*t946;
t1164 = t42.*t946;
t1165 = t43.*t946;
t1166 = -t1153;
t1167 = t45.*t946;
t1170 = -t1157;
t1173 = -t1163;
t1177 = -t1171;
t1182 = t59.*t946;
t1187 = t62.*t946;
t1190 = -t1189;
t1192 = -t1191;
t1194 = -t1193;
t1204 = -t1203;
t1247 = t192+t564+t669;
t1248 = t189+t190+t361+t373;
t1273 = t197+t204+t562+t574+t676;
t1274 = t194+t202+t567+t572+t674;
t1275 = t946.*t1272;
t378 = -t376;
t655 = -t647;
t857 = -t809;
t882 = -t835;
t953 = t937.^2;
t966 = t4.*t950;
t967 = t8.*t950;
t969 = -t963;
t1084 = t188+t375;
t1185 = t962.*(-3.146556677756745e-13);
t1217 = t808+t832;
t1218 = t807+t835;
t1226 = -t3.*(t809-t832);
t1228 = -t7.*(t809-t832);
t1251 = t339+t377+t381+t382;
t1262 = -t4.*(t7.*(t809-t832)+(t3.*t30.*t72.*(t26-t27))./8.112963841460668e+31);
t1263 = -t8.*(t7.*(t809-t832)+(t3.*t30.*t72.*(t26-t27))./8.112963841460668e+31);
t1268 = t4.*(t7.*(t809-t832)+(t3.*t30.*t72.*(t26-t27))./8.112963841460668e+31);
t1276 = -t1275;
t1283 = t77+t538+t1274;
t1345 = t80+t203+t210+t221+t550+t559+t573+t575+t580+t681+t683;
t1346 = t81+t209+t211+t222+t551+t555+t576+t578+t581+t677+t684;
t1440 = t199+t212+t214+t215+t220+t225+t235+t252+t254+t263+t274+t301+t310+t387+t393+t396+t406+t414+t420+t432+t450+t453+t454+t464+t466+t470+t477+t495+t500+t508+t515+t533+t535+t541+t543+t554+t557+t682+t686+t687+t688+t693+t700+t703+t704+t706+t710+t715+t716+t719+t723+t746+t750+t751+t754+t760+t765+t795+t802+t822+t834+t846+t851+t864+t873+t876+t879+t881+t889+t892+t894+t897+t904+t912+t914+t919+t939+t941+t944+t948+t954+t956+t989+t1015+t1024+t1027+t1049+t1051+t1057+t1067+t1069+t1092+t1096+t1099;
t1441 = t213+t228+t239+t243+t244+t250+t256+t259+t265+t266+t279+t293+t299+t304+t313+t314+t323+t359+t391+t401+t409+t413+t419+t425+t435+t437+t452+t459+t461+t463+t469+t472+t476+t489+t494+t497+t499+t507+t514+t546+t548+t560+t679+t689+t696+t701+t707+t714+t717+t718+t721+t725+t731+t734+t739+t741+t744+t745+t747+t748+t753+t758+t759+t766+t768+t771+t772+t788+t789+t791+t794+t800+t813+t828+t830+t840+t842+t850+t861+t863+t875+t880+t884+t888+t896+t903+t906+t909+t915+t918+t920+t922+t947+t958+t961+t982+t987+t990+t992+t1000+t1008+t1013+t1022+t1025+t1031+t1039+t1043+t1045+t1046+t1053+t1061+t1062+t1065+t1072+t1073+t1078+t1093+t1097+t1100;
et1 = t218+t232+t234+t246+t248+t251+t257+t258+t260+t261+t267+t268+t278+t282+t287+t289+t291+t292+t294+t295+t296+t298+t303+t305+t307+t315+t316+t319+t321+t322+t326+t327+t328+t329+t331+t332+t336+t337+t341+t343+t344+t345+t346+t347+t348+t349+t351+t353+t354+t365+t366+t374+t388+t402+t407+t412+t426+t429+t433+t434+t436+t442+t446+t449+t451+t460+t467+t468+t473+t474+t478+t480+t486+t493+t498+t503+t505+t506+t509+t518+t520+t522+t534+t540+t544+t545+t553+t558+t577+t582+t584+t585+t587+t590+t593+t594+t596+t597+t598+t600+t602+t604+t605+t606+t607+t611+t612+t615+t616+t617+t619+t620+t621+t622+t624+t625+t626+t627+t629+t633+t635+t636+t637+t638+t639+t640+t641+t642+t648+t650+t651+t652+t654+t657+t658+t662+t663+t664+t667+t673+t680+t699+t755+t756+t761+t769+t770+t775+t778+t780+t793+t797+t803+t811+t812+t815+t817+t820+t823+t831+t837+t849+t853+t856+t858+t862+t866+t868+t869+t874+t885+t887+t891+t893+t895+t899+t900+t901+t907+t911+t913+t916+t921+t930+t936+t940+t943+t945+t949+t957+t964+t968+t970+t974+t975+t978+t988+t991+t999+t1002;
et2 = t1009+t1011+t1012+t1019+t1023+t1032+t1041+t1042+t1044+t1047+t1048+t1059+t1063+t1064+t1066+t1071+t1079+t1080+t1089+t1094+t1101+t1102+t1105+t1106+t1107+t1108+t1110+t1112+t1113+t1114+t1115+t1116+t1118+t1120+t1121+t1123+t1124+t1126+t1128+t1129+t1131+t1134+t1136+t1139+t1140+t1141+t1142+t1143+t1144+t1145+t1152+t1155+t1158+t1159+t1160+t1166+t1169+t1170+t1172+t1173+t1175+t1176+t1177+t1178+t1179+t1180+t1181+t1183+t1190+t1192+t1194+t1195+t1197+t1199+t1200+t1201+t1202+t1204;
et3 = 3.626861556360138e-4;
t1442 = et1+et2+et3;
t1087 = t187+t378;
t1091 = t3.*t1084;
t1174 = t966.*4.20092050615074e-6;
t1184 = t966.*3.146556677756745e-13;
t1188 = t966.*4.126305279697715e-13;
t1205 = t953.*4.040985049072001e-70;
t1208 = t530+t966;
t1209 = t537+t967;
t1211 = -t5.*(t529-t967);
t1212 = -t9.*(t529-t967);
t1220 = t832+t857;
t1221 = t806+t882;
t1222 = t3.*t1218;
t1223 = t4.*t1217;
t1224 = t7.*t1218;
t1225 = t8.*t1217;
t1234 = t5.*(t529-t967).*(-1.744166498897461e-6);
t1235 = -t42.*(t529-t967);
t1236 = -t43.*(t529-t967);
t1237 = t9.*(t529-t967).*(-3.383302988283333e-6);
t1238 = t5.*(t529-t967).*1.744166498897461e-6;
t1239 = t5.*(t529-t967).*1.246862701090643e-6;
t1241 = t9.*(t529-t967).*(-3.146556677756745e-13);
t1243 = t9.*(t529-t967).*3.146556677756745e-13;
t1245 = t5.*(t529-t967).*(-4.126305279697715e-13);
t1246 = t5.*(t529-t967).*4.126305279697715e-13;
t1254 = t653+t1228;
t1258 = t660+t1226;
t1288 = -t1270.*(t529-t967);
t1329 = -t1248.*(t963+t5.*(t529-t967));
t1337 = t1248.*(t963+t5.*(t529-t967)).*(-7.26735e-3);
t1338 = t1248.*(t963+t5.*(t529-t967)).*7.26735e-3;
t1339 = t1248.*(t963+t5.*(t529-t967)).*(-7.26350610236655e-5);
t1341 = t1248.*(t963+t5.*(t529-t967)).*(-1.40259855e-11);
t1342 = t1248.*(t963+t5.*(t529-t967)).*1.40259855e-11;
t1098 = t3.*t1087;
t1186 = -t1184;
t1210 = t1208.^2;
t1213 = t504+t1091;
t1214 = (t475-t1091).^2;
t1227 = t4.*t1221;
t1229 = t8.*t1221;
t1252 = t646+t1224;
t1253 = t655+t1222;
t1257 = (t647-t1222).^2;
t1259 = -t5.*(t647-t1222);
t1260 = -t9.*(t647-t1222);
t1264 = t1258.^2;
t1265 = t962+t1212;
t1266 = t5.*t1258;
t1267 = t9.*t1258;
t1269 = t969+t1211;
t1277 = t1208.*t1248;
t1285 = -t1208.*(t963+t5.*(t529-t967));
t1286 = t1208.*(t963+t5.*(t529-t967));
t1287 = t1208.*t1271;
t1417 = t198+t333+t384+t423+t512+t519+t532+t685+t752+t785+t826+t839+t859+t925+t928+t935+t1021+t1081+t1086+t1161+t1164+t1188+t1236+t1238;
t1420 = t227+t241+t386+t394+t404+t424+t441+t465+t668+t695+t702+t711+t730+t814+t833+t860+t867+t886+t905+t1001+t1029+t1038+t1058+t1174+t1185+t1187+t1243+t1246;
t1215 = t510+t1098;
t1230 = t1210.*1.33637579258949e-4;
t1231 = t1210.*7.26350610236655e-5;
t1232 = t1210.*4.20092050615074e-6;
t1240 = t1210.*3.146556677756745e-13;
t1244 = t1210.*4.126305279697715e-13;
t1249 = t1214.*4.040985049072001e-70;
t1255 = t4.*t1252;
t1256 = t8.*t1252;
t1278 = -t1277;
t1279 = t1277.*1.33637579258949e-4;
t1280 = t1277.*7.26735e-3;
t1281 = t1277.*7.26350610236655e-5;
t1284 = t1208.*t1265;
t1295 = t1227+t1263;
t1297 = t1229+t1268;
t1302 = t1286.*(-7.26350610236655e-5);
t1304 = t1286.*7.26350610236655e-5;
t1305 = t1286.*(-1.246862701090643e-6);
t1307 = t1286.*(-1.744166498897461e-6);
t1308 = t1286.*1.246862701090643e-6;
t1309 = t1286.*1.744166498897461e-6;
t1313 = t1286.*(-1.40259855e-11);
t1314 = t1286.*(-4.126305279697715e-13);
t1315 = t1286.*1.40259855e-11;
t1316 = t1286.*4.126305279697715e-13;
t1328 = t1248.*t1265;
t1344 = t959+t1257+t1264;
t1416 = t191+t342+t379+t397+t511+t523+t531+t671+t728+t787+t810+t816+t821+t927+t929+t934+t984+t1077+t1085+t1165+t1167+t1186+t1237+t1239;
t1216 = t1215.^2;
t1233 = -t1231;
t1242 = -t1240;
t1261 = -t1255;
t1282 = -t1281;
t1289 = t1223+t1256;
t1294 = t1284.*1.33637579258949e-4;
t1298 = t1284.*1.246862701090643e-6;
t1299 = t1284.*3.383302988283333e-6;
t1300 = t5.*t1295;
t1301 = t9.*t1295;
t1303 = t1297.^2;
t1310 = t1284.*3.146556677756745e-13;
t1311 = t1284.*1.40259855e-11;
t1330 = -t1328;
t1334 = t1328.*1.33637579258949e-4;
t1335 = t1328.*7.26735e-3;
t1340 = t1328.*1.40259855e-11;
t1352 = t1251.*t1297.*(t26-t27).*(-7.596454196607839e-68);
t1358 = t1251.*t1297.*(t26-t27).*(-1.015171749786156e-71);
t1359 = t1251.*t1297.*(t26-t27).*(-5.520609140571798e-70);
t1360 = t1251.*t1297.*(t26-t27).*(-5.517689141340903e-72);
t1361 = t1251.*t1297.*(t26-t27).*1.015171749786156e-71;
t1362 = t1251.*t1297.*(t26-t27).*5.520609140571798e-70;
t1250 = t1216.*4.040985049072001e-70;
t1290 = t1225+t1261;
t1291 = t5.*t1289;
t1292 = t9.*t1289;
t1306 = -t1301;
t1312 = -t1310;
t1321 = t1303.*1.33637579258949e-4;
t1322 = t1303.*7.26350610236655e-5;
t1324 = t1303.*4.20092050615074e-6;
t1331 = t1303.*3.146556677756745e-13;
t1333 = t1303.*4.126305279697715e-13;
t1336 = -t1334;
t1349 = t1267+t1300;
t1293 = t1290.^2;
t1296 = -t1292;
t1323 = -t1322;
t1332 = -t1331;
t1343 = t1205+t1249+t1250;
t1347 = t1260+t1291;
t1350 = t1266+t1306;
t1351 = (t47.*t1251.*t1290)./1.316403645856965e+67;
t1353 = t47.*t1251.*t1290.*1.015171749786156e-71;
t1354 = t47.*t1251.*t1290.*5.520609140571798e-70;
t1355 = t47.*t1251.*t1290.*5.517689141340903e-72;
t1364 = t47.*t1251.*(t1292+t5.*(t647-t1222)).*(-7.596454196607839e-68);
t1365 = t1251.*t1349.*(t26-t27).*(-7.596454196607839e-68);
t1370 = t47.*t1251.*(t1292+t5.*(t647-t1222)).*(-1.015171749786156e-71);
t1371 = t47.*t1251.*(t1292+t5.*(t647-t1222)).*(-5.520609140571798e-70);
t1372 = t47.*t1251.*(t1292+t5.*(t647-t1222)).*5.520609140571798e-70;
t1375 = t1251.*t1349.*(t26-t27).*(-5.520609140571798e-70);
t1376 = t47.*t1251.*(t1292+t5.*(t647-t1222)).*(-1.065477564130357e-78);
t1377 = t1251.*t1349.*(t26-t27).*(-5.517689141340903e-72);
t1378 = t1251.*t1349.*(t26-t27).*5.520609140571798e-70;
t1379 = t47.*t1251.*(t1292+t5.*(t647-t1222)).*1.065477564130357e-78;
t1383 = t1251.*t1349.*(t26-t27).*(-1.065477564130357e-78);
t1384 = t1251.*t1349.*(t26-t27).*1.065477564130357e-78;
t1389 = -t1290.*(t1292+t5.*(t647-t1222));
t1390 = t1297.*t1349;
t1393 = t1290.*(t1292+t5.*(t647-t1222)).*(-1.33637579258949e-4);
t1396 = t1290.*(t1292+t5.*(t647-t1222)).*(-1.246862701090643e-6);
t1397 = t1290.*(t1292+t5.*(t647-t1222)).*(-3.383302988283333e-6);
t1400 = t1290.*(t1292+t5.*(t647-t1222)).*(-3.146556677756745e-13);
t1401 = t1290.*(t1292+t5.*(t647-t1222)).*(-1.40259855e-11);
t1402 = t1290.*(t1292+t5.*(t647-t1222)).*3.146556677756745e-13;
t1317 = t1293.*1.33637579258949e-4;
t1318 = t1293.*7.26350610236655e-5;
t1320 = t1293.*4.20092050615074e-6;
t1325 = t1293.*3.146556677756745e-13;
t1327 = t1293.*4.126305279697715e-13;
t1348 = t1259+t1296;
t1356 = -t1353;
t1357 = -t1354;
t1363 = (t47.*t1251.*t1347)./1.316403645856965e+67;
t1366 = t1251.*t1350.*(t26-t27).*(-7.596454196607839e-68);
t1367 = t47.*t1251.*t1347.*5.520609140571798e-70;
t1368 = t47.*t1251.*t1347.*5.517689141340903e-72;
t1373 = t47.*t1251.*t1347.*1.065477564130357e-78;
t1380 = t1251.*t1350.*(t26-t27).*(-1.015171749786156e-71);
t1381 = t1251.*t1350.*(t26-t27).*(-5.520609140571798e-70);
t1382 = t1251.*t1350.*(t26-t27).*5.520609140571798e-70;
t1385 = t1251.*t1350.*(t26-t27).*(-1.065477564130357e-78);
t1386 = t1251.*t1350.*(t26-t27).*1.065477564130357e-78;
t1387 = t1210+t1293+t1303;
t1388 = t1290.*t1347;
t1391 = t1297.*t1350;
t1403 = t1390.*7.26350610236655e-5;
t1405 = t1390.*1.744166498897461e-6;
t1406 = t1390.*1.246862701090643e-6;
t1409 = t1390.*1.40259855e-11;
t1410 = t1390.*4.126305279697715e-13;
t1414 = t1278+t1351+t1352;
t1319 = -t1318;
t1326 = -t1325;
t1369 = -t1367;
t1374 = -t1373;
t1392 = t1388.*7.26350610236655e-5;
t1394 = t1388.*1.744166498897461e-6;
t1395 = t1388.*1.246862701090643e-6;
t1398 = t1388.*1.40259855e-11;
t1399 = t1388.*4.126305279697715e-13;
t1404 = t1391.*1.33637579258949e-4;
t1407 = t1391.*1.246862701090643e-6;
t1408 = t1391.*3.383302988283333e-6;
t1411 = t1391.*3.146556677756745e-13;
t1412 = t1391.*1.40259855e-11;
t1415 = t85+t87+t107+t113+t114+t140+t1280+t1357+t1362;
t1418 = t1329+t1363+t1365;
t1419 = t1330+t1364+t1366;
t1421 = t78+t88+t158+t170+t178+t1335+t1372+t1382;
t1423 = t1284+t1389+t1391;
t1424 = t1286+t1388+t1390;
t1428 = t108+t132+t136+t138+t146+t152+t160+t167+t1282+t1340+t1355+t1360+t1379+t1386;
t1433 = t96+t133+t156+t166+t168+t172+t175+t177+t1336+t1339+t1368+t1370+t1377+t1380;
et4 = t90+t119+t150+t161-t168+t169-t172-t177+t1334-t1368+t1248.*(t963+t5.*(t529-t967)).*7.26350610236655e-5+t47.*t1251.*(t1292+t5.*(t647-t1222)).*1.015171749786156e-71;
et5 = t1251.*t1349.*(t26-t27).*5.517689141340903e-72;
et6 = t1251.*t1350.*(t26-t27).*1.015171749786156e-71;
t1434 = -t1208.*(et4+et5+et6);
et7 = t90+t119+t150+t161-t168+t169-t172-t177+t1334-t1368+t1248.*(t963+t5.*(t529-t967)).*7.26350610236655e-5+t47.*t1251.*(t1292+t5.*(t647-t1222)).*1.015171749786156e-71;
et8 = t1251.*t1349.*(t26-t27).*5.517689141340903e-72;
et9 = t1251.*t1350.*(t26-t27).*1.015171749786156e-71;
t1435 = t1208.*(et7+et8+et9);
t1413 = -t1411;
t1422 = t89+t106+t159+t164+t179+t1338+t1369+t1378;
t1425 = t1230+t1315+t1317+t1321+t1398+t1409;
t1426 = t1233+t1311+t1319+t1323+t1401+t1412;
t1427 = t115+t120+t124+t130+t135+t144+t151+t162+t1279+t1342+t1356+t1361+t1374+t1384;
t1431 = -t1428.*(t963+t5.*(t529-t967));
t1432 = t1428.*(t963+t5.*(t529-t967));
t1436 = t1294+t1304+t1392+t1393+t1403+t1404;
t1437 = t1242+t1299+t1308+t1326+t1332+t1395+t1397+t1406+t1408;
t1438 = t1244+t1298+t1309+t1327+t1333+t1394+t1396+t1405+t1407;
t1429 = t1265.*t1427;
t1439 = t1232+t1312+t1316+t1320+t1324+t1399+t1402+t1410+t1413;
t1430 = -t1429;
et10 = t2.*2.821008266589887e-4;
et11 = t6.*9.795760612003476e-4+t218+t232+t234+t246+t248+t251+t257+t258+t260+t261+t267+t268+t278+t282+t287+t289+t291+t292+t294+t295+t296+t298+t303+t305+t307+t315+t316+t319+t321+t322;
et12 = t326+t327+t328+t329+t331+t332+t336+t337+t341+t343+t344+t345+t346+t347+t348+t349+t351+t353+t354+t365+t366+t374+t402+t442+t449+t451+t474+t486+t503+t505+t518+t522+t544+t553+t577+t582+t584+t585+t587+t590+t594+t597+t598+t600+t602+t604+t605+t606+t607+t611+t612+t615+t616+t617+t619+t620+t621+t622+t624+t625+t626+t627+t629+t633+t635+t636+t637+t638+t639+t640+t641+t642+t648+t650+t651+t652+t654+t657+t658+t662+t663+t664+t667+t673+t680+t699+t755+t756+t761+t770+t775+t780+t793+t811+t820+t823+t837+t856+t858+t862+t868+t869+t891+t901+t911+t916+t921+t930+t936+t945+t964+t968+t970+t974+t978+t999+t1019+t1032+t1041+t1071+t1089+t1102+t1105+t1106+t1107+t1108+t1110+t1112+t1113+t1114+t1115+t1116+t1118+t1120+t1121+t1123+t1124+t1126+t1128+t1129+t1131+t1134+t1136+t1139+t1140+t1141+t1142+t1143+t1144+t1145+t1152+t1155+t1158+t1159+t1160+t1166+t1169+t1170+t1172+t1173+t1175+t1176+t1177+t1178+t1179+t1180+t1181+t1183+t1190+t1192+t1194+t1195+t1197+t1199+t1200+t1201+t1202+t1204;
et13 = t2.*t3.*7.556062069816369e-6;
et14 = t2.*t4.*2.793386635594598e-6;
et15 = t2.*t7.*(-8.334431886523961e-9);
et16 = t3.*t6.*3.116899618889927e-5;
et17 = t2.*t8.*3.593132588990334e-6;
et18 = t4.*t6.*1.152280865277303e-5;
et19 = t6.*t7.*(-3.437979642139428e-8);
et20 = t6.*t8.*1.482178612849474e-5;
et21 = t2.*t71.*3.95755796128007e-4;
et22 = t2.*t74.*(-1.853092799186148e-5);
et23 = t2.*t75.*2.043984759722906e-8;
et24 = t6.*t71.*(-9.594005985658975e-5);
et25 = t6.*t74.*4.492311567212771e-6;
et26 = t6.*t75.*(-4.955076390854535e-9);
et27 = t2.*t3.*t5.*3.236065815824815e-6;
et28 = t2.*t4.*t5.*3.539761430212882e-6;
et29 = t2.*t4.*t7.*6.043644226648326e-6;
et30 = t2.*t3.*t9.*(-5.953874008704457e-6);
et31 = t3.*t5.*t6.*1.334887434069505e-5;
et32 = t2.*t4.*t9.*1.923940772636472e-6;
et33 = t4.*t5.*t6.*1.460162840226632e-5;
et34 = t2.*t7.*t8.*(-4.698472598739189e-6);
et35 = t4.*t6.*t7.*2.493022451733813e-5;
et36 = t3.*t6.*t9.*(-2.455991951519339e-5);
et37 = t4.*t6.*t9.*7.93631683486574e-6;
et38 = t6.*t7.*t8.*(-1.938134879923087e-5);
et39 = t2.*t4.*t71.*1.938134879923087e-5;
et40 = t2.*t4.*t75.*(-1.482178612849474e-5);
et41 = t2.*t5.*t74.*(-7.93631683486574e-6);
et42 = t2.*t8.*t71.*2.493022451733813e-5;
et43 = t4.*t6.*t71.*(-4.698472598739189e-6);
et44 = t2.*t8.*t75.*1.152280865277303e-5;
et45 = t2.*t9.*t74.*1.460162840226632e-5;
et46 = t4.*t6.*t75.*3.593132588990334e-6;
et47 = t5.*t6.*t74.*1.923940772636472e-6;
et48 = t6.*t8.*t71.*(-6.043644226648326e-6);
et49 = t6.*t8.*t75.*(-2.793386635594598e-6);
et50 = t6.*t9.*t74.*(-3.539761430212882e-6);
et51 = t2.*t30.*t72.*4.096256460969035e-28;
et52 = t6.*t30.*t72.*(-9.930242182130862e-29);
et53 = t2.*t5.*t7.*t8.*(-5.953874008704457e-6);
et54 = t2.*t7.*t8.*t9.*(-3.236065815824815e-6);
et55 = t5.*t6.*t7.*t8.*(-2.455991951519339e-5);
et56 = t6.*t7.*t8.*t9.*(-1.334887434069505e-5);
et57 = t2.*t4.*t5.*t71.*2.455991951519339e-5;
et58 = t2.*t4.*t9.*t71.*1.334887434069505e-5;
et59 = t4.*t5.*t6.*t71.*(-5.953874008704457e-6);
H = ft_3({et10,et11,et12,et13,et14,et15,et16,et17,et18,et19,et20,et21,et22,et23,et24,et25,et26,et27,et28,et29,et30,et31,et32,et33,et34,et35,et36,et37,et38,et39,et40,et41,et42,et43,et44,et45,et46,et47,et48,et49,et50,et51,et52,et53,et54,et55,et56,et57,et58,et59,t1000,t1001,t1007,t101,t1010,t1019,t102,t1022,t1028,t1029,t1030,t1032,t1035,t1036,t1037,t1038,t1039,t1040,t1041,t1043,t1050,t1058,t1065,t1071,t1073,t1077,t1078,t1082,t1089,t1090,t1100,t1102,t1105,t1106,t1107,t1108,t1110,t1112,t1113,t1114,t1115,t1116,t1118,t1120,t1121,t1123,t1124,t1126,t1128,t1129,t1130,t1131,t1134,t1136,t1138,t1139,t1140,t1141,t1142,t1143,t1144,t1145,t1147,t1152,t1154,t1155,t1158,t1159,t1160,t1166,t1168,t1169,t1170,t1172,t1173,t1175,t1176,t1177,t1178,t1179,t1180,t1181,t1183,t1184,t119,t1190,t1192,t1194,t1195,t1197,t1198,t1199,t1200,t1201,t1202,t1204,t1206,t1207,t1208,t121,t1214,t1216,t1219,t1222,t1231,t1235,t1240,t1247,t1248,t1251,t1265,t1272,t1273,t1274,t1276,t1277,t1283,t1284,t1286,t1287,t1288,t1290,t1292,t1297,t1299,t1308,t1311,t1318,t1322,t1326,t1328,t1332,t1334,t134,t1343,t1344,t1345,t1346,t1349,t1350,t1351,t1363,t1368,t1387,t1388,t1390,t1391,t1395,t1397,t14,t1406,t1408,t141,t1412,t1415,t1416,t1417,t1420,t1421,t1422,t1423,t1424,t1425,t1427,t1428,t1430,t1432,t1435,t1436,t1438,t1439,t1440,t1441,t1442,t149,t15,t150,t153,t154,t16,t160,t161,t163,t168,t169,t17,t171,t172,t177,t18,t180,t181,t184,t186,t19,t191,t196,t2,t20,t200,t21,t213,t217,t218,t219,t227,t228,t232,t233,t234,t237,t239,t240,t241,t243,t244,t246,t248,t250,t251,t255,t256,t257,t258,t259,t26,t260,t261,t262,t265,t266,t267,t268,t27,t273,t278,t279,t282,t287,t288,t289,t291,t292,t293,t294,t295,t296,t298,t299,t3,t30,t302,t303,t304,t305,t307,t313,t314,t315,t316,t319,t321,t322,t323,t326,t327,t328,t329,t331,t332,t334,t336,t337,t341,t343,t344,t345,t346,t347,t348,t349,t35,t351,t353,t354,t355,t356,t357,t359,t362,t364,t365,t366,t368,t374,t379,t38,t380,t383,t385,t386,t391,t394,t395,t397,t4,t402,t404,t405,t408,t409,t415,t416,t419,t424,t425,t427,t441,t442,t447,t448,t449,t451,t455,t458,t461,t463,t465,t47,t471,t474,t476,t479,t486,t496,t5,t501,t503,t505,t511,t518,t521,t522,t524,t528,t529,t530,t544,t548,t553,t566,t568,t569,t570,t577,t579,t582,t583,t584,t585,t586,t587,t588,t590,t591,t594,t595,t597,t598,t6,t600,t602,t603,t604,t605,t606,t607,t611,t612,t615,t616,t617,t619,t62,t620,t621,t622,t623,t624,t625,t626,t627,t629,t633,t635,t636,t637,t638,t639,t640,t641,t642,t647,t648,t650,t651,t652,t654,t657,t658,t662,t663,t664,t667,t668,t670,t671,t672,t673,t679,t680,t687,t689,t695,t696,t699,t7,t701,t702,t707,t71,t711,t712,t714,t717,t718,t72,t720,t721,t725,t730,t731,t734,t736,t739,t74,t741,t744,t745,t747,t748,t75,t753,t755,t756,t758,t759,t761,t766,t767,t770,t771,t772,t773,t775,t779,t780,t786,t789,t791,t793,t796,t8,t801,t811,t814,t816,t820,t821,t823,t828,t829,t833,t837,t840,t841,t843,t845,t852,t854,t856,t858,t860,t861,t862,t863,t867,t868,t869,t877,t886,t890,t891,t9,t90,t901,t903,t905,t906,t911,t915,t916,t918,t920,t921,t922,t923,t926,t930,t931,t936,t945,t946,t953,t961,t962,t963,t964,t966,t967,t968,t970,t971,t974,t978,t983,t984,t993,t999});
end
function H = ft_3(ct)
et10 = ct{1};
et11 = ct{2};
et12 = ct{3};
et13 = ct{4};
et14 = ct{5};
et15 = ct{6};
et16 = ct{7};
et17 = ct{8};
et18 = ct{9};
et19 = ct{10};
et20 = ct{11};
et21 = ct{12};
et22 = ct{13};
et23 = ct{14};
et24 = ct{15};
et25 = ct{16};
et26 = ct{17};
et27 = ct{18};
et28 = ct{19};
et29 = ct{20};
et30 = ct{21};
et31 = ct{22};
et32 = ct{23};
et33 = ct{24};
et34 = ct{25};
et35 = ct{26};
et36 = ct{27};
et37 = ct{28};
et38 = ct{29};
et39 = ct{30};
et40 = ct{31};
et41 = ct{32};
et42 = ct{33};
et43 = ct{34};
et44 = ct{35};
et45 = ct{36};
et46 = ct{37};
et47 = ct{38};
et48 = ct{39};
et49 = ct{40};
et50 = ct{41};
et51 = ct{42};
et52 = ct{43};
et53 = ct{44};
et54 = ct{45};
et55 = ct{46};
et56 = ct{47};
et57 = ct{48};
et58 = ct{49};
et59 = ct{50};
t1000 = ct{51};
t1001 = ct{52};
t1007 = ct{53};
t101 = ct{54};
t1010 = ct{55};
t1019 = ct{56};
t102 = ct{57};
t1022 = ct{58};
t1028 = ct{59};
t1029 = ct{60};
t1030 = ct{61};
t1032 = ct{62};
t1035 = ct{63};
t1036 = ct{64};
t1037 = ct{65};
t1038 = ct{66};
t1039 = ct{67};
t1040 = ct{68};
t1041 = ct{69};
t1043 = ct{70};
t1050 = ct{71};
t1058 = ct{72};
t1065 = ct{73};
t1071 = ct{74};
t1073 = ct{75};
t1077 = ct{76};
t1078 = ct{77};
t1082 = ct{78};
t1089 = ct{79};
t1090 = ct{80};
t1100 = ct{81};
t1102 = ct{82};
t1105 = ct{83};
t1106 = ct{84};
t1107 = ct{85};
t1108 = ct{86};
t1110 = ct{87};
t1112 = ct{88};
t1113 = ct{89};
t1114 = ct{90};
t1115 = ct{91};
t1116 = ct{92};
t1118 = ct{93};
t1120 = ct{94};
t1121 = ct{95};
t1123 = ct{96};
t1124 = ct{97};
t1126 = ct{98};
t1128 = ct{99};
t1129 = ct{100};
t1130 = ct{101};
t1131 = ct{102};
t1134 = ct{103};
t1136 = ct{104};
t1138 = ct{105};
t1139 = ct{106};
t1140 = ct{107};
t1141 = ct{108};
t1142 = ct{109};
t1143 = ct{110};
t1144 = ct{111};
t1145 = ct{112};
t1147 = ct{113};
t1152 = ct{114};
t1154 = ct{115};
t1155 = ct{116};
t1158 = ct{117};
t1159 = ct{118};
t1160 = ct{119};
t1166 = ct{120};
t1168 = ct{121};
t1169 = ct{122};
t1170 = ct{123};
t1172 = ct{124};
t1173 = ct{125};
t1175 = ct{126};
t1176 = ct{127};
t1177 = ct{128};
t1178 = ct{129};
t1179 = ct{130};
t1180 = ct{131};
t1181 = ct{132};
t1183 = ct{133};
t1184 = ct{134};
t119 = ct{135};
t1190 = ct{136};
t1192 = ct{137};
t1194 = ct{138};
t1195 = ct{139};
t1197 = ct{140};
t1198 = ct{141};
t1199 = ct{142};
t1200 = ct{143};
t1201 = ct{144};
t1202 = ct{145};
t1204 = ct{146};
t1206 = ct{147};
t1207 = ct{148};
t1208 = ct{149};
t121 = ct{150};
t1214 = ct{151};
t1216 = ct{152};
t1219 = ct{153};
t1222 = ct{154};
t1231 = ct{155};
t1235 = ct{156};
t1240 = ct{157};
t1247 = ct{158};
t1248 = ct{159};
t1251 = ct{160};
t1265 = ct{161};
t1272 = ct{162};
t1273 = ct{163};
t1274 = ct{164};
t1276 = ct{165};
t1277 = ct{166};
t1283 = ct{167};
t1284 = ct{168};
t1286 = ct{169};
t1287 = ct{170};
t1288 = ct{171};
t1290 = ct{172};
t1292 = ct{173};
t1297 = ct{174};
t1299 = ct{175};
t1308 = ct{176};
t1311 = ct{177};
t1318 = ct{178};
t1322 = ct{179};
t1326 = ct{180};
t1328 = ct{181};
t1332 = ct{182};
t1334 = ct{183};
t134 = ct{184};
t1343 = ct{185};
t1344 = ct{186};
t1345 = ct{187};
t1346 = ct{188};
t1349 = ct{189};
t1350 = ct{190};
t1351 = ct{191};
t1363 = ct{192};
t1368 = ct{193};
t1387 = ct{194};
t1388 = ct{195};
t1390 = ct{196};
t1391 = ct{197};
t1395 = ct{198};
t1397 = ct{199};
t14 = ct{200};
t1406 = ct{201};
t1408 = ct{202};
t141 = ct{203};
t1412 = ct{204};
t1415 = ct{205};
t1416 = ct{206};
t1417 = ct{207};
t1420 = ct{208};
t1421 = ct{209};
t1422 = ct{210};
t1423 = ct{211};
t1424 = ct{212};
t1425 = ct{213};
t1427 = ct{214};
t1428 = ct{215};
t1430 = ct{216};
t1432 = ct{217};
t1435 = ct{218};
t1436 = ct{219};
t1438 = ct{220};
t1439 = ct{221};
t1440 = ct{222};
t1441 = ct{223};
t1442 = ct{224};
t149 = ct{225};
t15 = ct{226};
t150 = ct{227};
t153 = ct{228};
t154 = ct{229};
t16 = ct{230};
t160 = ct{231};
t161 = ct{232};
t163 = ct{233};
t168 = ct{234};
t169 = ct{235};
t17 = ct{236};
t171 = ct{237};
t172 = ct{238};
t177 = ct{239};
t18 = ct{240};
t180 = ct{241};
t181 = ct{242};
t184 = ct{243};
t186 = ct{244};
t19 = ct{245};
t191 = ct{246};
t196 = ct{247};
t2 = ct{248};
t20 = ct{249};
t200 = ct{250};
t21 = ct{251};
t213 = ct{252};
t217 = ct{253};
t218 = ct{254};
t219 = ct{255};
t227 = ct{256};
t228 = ct{257};
t232 = ct{258};
t233 = ct{259};
t234 = ct{260};
t237 = ct{261};
t239 = ct{262};
t240 = ct{263};
t241 = ct{264};
t243 = ct{265};
t244 = ct{266};
t246 = ct{267};
t248 = ct{268};
t250 = ct{269};
t251 = ct{270};
t255 = ct{271};
t256 = ct{272};
t257 = ct{273};
t258 = ct{274};
t259 = ct{275};
t26 = ct{276};
t260 = ct{277};
t261 = ct{278};
t262 = ct{279};
t265 = ct{280};
t266 = ct{281};
t267 = ct{282};
t268 = ct{283};
t27 = ct{284};
t273 = ct{285};
t278 = ct{286};
t279 = ct{287};
t282 = ct{288};
t287 = ct{289};
t288 = ct{290};
t289 = ct{291};
t291 = ct{292};
t292 = ct{293};
t293 = ct{294};
t294 = ct{295};
t295 = ct{296};
t296 = ct{297};
t298 = ct{298};
t299 = ct{299};
t3 = ct{300};
t30 = ct{301};
t302 = ct{302};
t303 = ct{303};
t304 = ct{304};
t305 = ct{305};
t307 = ct{306};
t313 = ct{307};
t314 = ct{308};
t315 = ct{309};
t316 = ct{310};
t319 = ct{311};
t321 = ct{312};
t322 = ct{313};
t323 = ct{314};
t326 = ct{315};
t327 = ct{316};
t328 = ct{317};
t329 = ct{318};
t331 = ct{319};
t332 = ct{320};
t334 = ct{321};
t336 = ct{322};
t337 = ct{323};
t341 = ct{324};
t343 = ct{325};
t344 = ct{326};
t345 = ct{327};
t346 = ct{328};
t347 = ct{329};
t348 = ct{330};
t349 = ct{331};
t35 = ct{332};
t351 = ct{333};
t353 = ct{334};
t354 = ct{335};
t355 = ct{336};
t356 = ct{337};
t357 = ct{338};
t359 = ct{339};
t362 = ct{340};
t364 = ct{341};
t365 = ct{342};
t366 = ct{343};
t368 = ct{344};
t374 = ct{345};
t379 = ct{346};
t38 = ct{347};
t380 = ct{348};
t383 = ct{349};
t385 = ct{350};
t386 = ct{351};
t391 = ct{352};
t394 = ct{353};
t395 = ct{354};
t397 = ct{355};
t4 = ct{356};
t402 = ct{357};
t404 = ct{358};
t405 = ct{359};
t408 = ct{360};
t409 = ct{361};
t415 = ct{362};
t416 = ct{363};
t419 = ct{364};
t424 = ct{365};
t425 = ct{366};
t427 = ct{367};
t441 = ct{368};
t442 = ct{369};
t447 = ct{370};
t448 = ct{371};
t449 = ct{372};
t451 = ct{373};
t455 = ct{374};
t458 = ct{375};
t461 = ct{376};
t463 = ct{377};
t465 = ct{378};
t47 = ct{379};
t471 = ct{380};
t474 = ct{381};
t476 = ct{382};
t479 = ct{383};
t486 = ct{384};
t496 = ct{385};
t5 = ct{386};
t501 = ct{387};
t503 = ct{388};
t505 = ct{389};
t511 = ct{390};
t518 = ct{391};
t521 = ct{392};
t522 = ct{393};
t524 = ct{394};
t528 = ct{395};
t529 = ct{396};
t530 = ct{397};
t544 = ct{398};
t548 = ct{399};
t553 = ct{400};
t566 = ct{401};
t568 = ct{402};
t569 = ct{403};
t570 = ct{404};
t577 = ct{405};
t579 = ct{406};
t582 = ct{407};
t583 = ct{408};
t584 = ct{409};
t585 = ct{410};
t586 = ct{411};
t587 = ct{412};
t588 = ct{413};
t590 = ct{414};
t591 = ct{415};
t594 = ct{416};
t595 = ct{417};
t597 = ct{418};
t598 = ct{419};
t6 = ct{420};
t600 = ct{421};
t602 = ct{422};
t603 = ct{423};
t604 = ct{424};
t605 = ct{425};
t606 = ct{426};
t607 = ct{427};
t611 = ct{428};
t612 = ct{429};
t615 = ct{430};
t616 = ct{431};
t617 = ct{432};
t619 = ct{433};
t62 = ct{434};
t620 = ct{435};
t621 = ct{436};
t622 = ct{437};
t623 = ct{438};
t624 = ct{439};
t625 = ct{440};
t626 = ct{441};
t627 = ct{442};
t629 = ct{443};
t633 = ct{444};
t635 = ct{445};
t636 = ct{446};
t637 = ct{447};
t638 = ct{448};
t639 = ct{449};
t640 = ct{450};
t641 = ct{451};
t642 = ct{452};
t647 = ct{453};
t648 = ct{454};
t650 = ct{455};
t651 = ct{456};
t652 = ct{457};
t654 = ct{458};
t657 = ct{459};
t658 = ct{460};
t662 = ct{461};
t663 = ct{462};
t664 = ct{463};
t667 = ct{464};
t668 = ct{465};
t670 = ct{466};
t671 = ct{467};
t672 = ct{468};
t673 = ct{469};
t679 = ct{470};
t680 = ct{471};
t687 = ct{472};
t689 = ct{473};
t695 = ct{474};
t696 = ct{475};
t699 = ct{476};
t7 = ct{477};
t701 = ct{478};
t702 = ct{479};
t707 = ct{480};
t71 = ct{481};
t711 = ct{482};
t712 = ct{483};
t714 = ct{484};
t717 = ct{485};
t718 = ct{486};
t72 = ct{487};
t720 = ct{488};
t721 = ct{489};
t725 = ct{490};
t730 = ct{491};
t731 = ct{492};
t734 = ct{493};
t736 = ct{494};
t739 = ct{495};
t74 = ct{496};
t741 = ct{497};
t744 = ct{498};
t745 = ct{499};
t747 = ct{500};
t748 = ct{501};
t75 = ct{502};
t753 = ct{503};
t755 = ct{504};
t756 = ct{505};
t758 = ct{506};
t759 = ct{507};
t761 = ct{508};
t766 = ct{509};
t767 = ct{510};
t770 = ct{511};
t771 = ct{512};
t772 = ct{513};
t773 = ct{514};
t775 = ct{515};
t779 = ct{516};
t780 = ct{517};
t786 = ct{518};
t789 = ct{519};
t791 = ct{520};
t793 = ct{521};
t796 = ct{522};
t8 = ct{523};
t801 = ct{524};
t811 = ct{525};
t814 = ct{526};
t816 = ct{527};
t820 = ct{528};
t821 = ct{529};
t823 = ct{530};
t828 = ct{531};
t829 = ct{532};
t833 = ct{533};
t837 = ct{534};
t840 = ct{535};
t841 = ct{536};
t843 = ct{537};
t845 = ct{538};
t852 = ct{539};
t854 = ct{540};
t856 = ct{541};
t858 = ct{542};
t860 = ct{543};
t861 = ct{544};
t862 = ct{545};
t863 = ct{546};
t867 = ct{547};
t868 = ct{548};
t869 = ct{549};
t877 = ct{550};
t886 = ct{551};
t890 = ct{552};
t891 = ct{553};
t9 = ct{554};
t90 = ct{555};
t901 = ct{556};
t903 = ct{557};
t905 = ct{558};
t906 = ct{559};
t911 = ct{560};
t915 = ct{561};
t916 = ct{562};
t918 = ct{563};
t920 = ct{564};
t921 = ct{565};
t922 = ct{566};
t923 = ct{567};
t926 = ct{568};
t930 = ct{569};
t931 = ct{570};
t936 = ct{571};
t945 = ct{572};
t946 = ct{573};
t953 = ct{574};
t961 = ct{575};
t962 = ct{576};
t963 = ct{577};
t964 = ct{578};
t966 = ct{579};
t967 = ct{580};
t968 = ct{581};
t970 = ct{582};
t971 = ct{583};
t974 = ct{584};
t978 = ct{585};
t983 = ct{586};
t984 = ct{587};
t993 = ct{588};
t999 = ct{589};
et60 = t2.*t5.*t8.*t75.*1.460162840226632e-5;
et61 = t4.*t6.*t9.*t71.*(-3.236065815824815e-6);
et62 = t2.*t8.*t9.*t75.*7.93631683486574e-6;
et63 = t5.*t6.*t8.*t75.*(-3.539761430212882e-6);
et64 = t6.*t8.*t9.*t75.*(-1.923940772636472e-6);
et65 = t2.*t3.*t30.*t72.*4.440555926585153e-24;
et66 = t2.*t7.*t30.*t72.*4.02584323234086e-21;
et67 = t3.*t6.*t30.*t72.*(-1.076490112239103e-24);
et68 = t6.*t7.*t30.*t72.*(-9.759544761262319e-22);
et69 = t2.*t3.*t4.*t30.*t72.*(-3.220032337442058e-21);
et70 = t2.*t3.*t8.*t30.*t72.*2.503329636416397e-21;
et71 = t3.*t4.*t6.*t30.*t72.*7.806078855113529e-22;
et72 = t2.*t5.*t7.*t30.*t72.*1.724164458109665e-21;
et73 = t3.*t6.*t8.*t30.*t72.*(-6.068631148509608e-22);
et74 = t2.*t7.*t9.*t30.*t72.*(-3.172203081801246e-21);
et75 = t5.*t6.*t7.*t30.*t72.*(-4.179760421250838e-22);
et76 = t6.*t7.*t9.*t30.*t72.*7.690130037838559e-22;
et77 = t2.*t3.*t5.*t8.*t30.*t72.*3.172203081801246e-21;
et78 = t2.*t3.*t8.*t9.*t30.*t72.*1.724164458109665e-21;
et79 = t3.*t5.*t6.*t8.*t30.*t72.*(-7.690130037838559e-22);
et80 = t3.*t6.*t8.*t9.*t30.*t72.*(-4.179760421250838e-22);
et81 = 1.453096634654864e-3;
et82 = t74.*3.87668616986977e-7+t383+t385+t408+t416+t583+t588+t591+t595+t603+t623+t1035+t1037+t1040+t1138+t1147+t1168;
et83 = t2.*t75.*4.395308215012666e-6;
et84 = t4.*t74.*(-1.200790562256725e-5);
et85 = t4.*t75.*(-6.359001115808088e-7)-t5.*t74.*2.10868590222219e-13;
et86 = t8.*t71.*1.069583140309415e-6+t5.*t75.*6.429626140715183e-6;
et87 = t6.*t75.*1.813078608102233e-5+t7.*t74.*3.40807331083027e-6;
et88 = t8.*t74.*9.33523109899656e-6-t9.*t74.*1.608000198040319e-13;
et89 = t9.*t75.*(-1.182954431201322e-5)-t17.*t74.*7.452372645815517e-7;
et90 = t30.*t72.*(-1.74829743798322e-20);
et91 = t2.*t4.*t74.*(-3.5155453823114e-6);
et92 = t4.*t5.*t71.*(-2.7046541903611e-13)+t2.*t5.*t75.*1.882396747564322e-6;
et93 = t2.*t8.*t74.*2.733068497907686e-6+t4.*t5.*t75.*2.227142959217101e-7;
et94 = t4.*t6.*t74.*(-1.4501736435025e-5);
et95 = t4.*t9.*t71.*3.546806877605634e-13-t5.*t8.*t71.*3.746051489620971e-7;
et96 = t2.*t9.*t75.*(-3.46332667728404e-6)-t4.*t8.*t74.*3.016314764575132e-7;
et97 = t5.*t6.*t75.*7.764946411068142e-6-t5.*t7.*t74.*1.378434177095879e-6;
et98 = t5.*t8.*t74.*1.182954431201322e-5-t4.*t9.*t75.*4.097607815548108e-7;
et99 = t5.*t8.*t75.*(-1.608000198040319e-13)+t6.*t8.*t74.*1.12739944177504e-5;
et100 = t8.*t9.*t71.*6.892170885479394e-7-t6.*t9.*t75.*1.428633261714363e-5;
et101 = t7.*t9.*t74.*(-7.492102979241942e-7)+t8.*t9.*t74.*6.429626140715183e-6;
et102 = t8.*t16.*t71.*(-2.139166280618831e-6)+t5.*t17.*t74.*4.217371804444381e-13;
et103 = t4.*t18.*t75.*1.274380648825446e-6-t8.*t18.*t71.*2.143506553146841e-6;
et104 = t7.*t17.*t74.*(-5.073437414621283e-7)-t7.*t18.*t74.*2.817872251232979e-6;
et105 = t9.*t17.*t74.*3.216000396080637e-13;
et106 = t2.*t30.*t72.*(-5.325743171835082e-21);
et107 = t4.*t30.*t72.*(-1.185912239144439e-21);
et108 = t5.*t30.*t72.*7.82072115054759e-23;
et109 = t6.*t30.*t72.*(-2.196885984950864e-20);
et110 = t7.*t30.*t72.*3.845355261323178e-23;
et111 = t8.*t30.*t72.*(-1.525438641344884e-21);
et112 = t9.*t30.*t72.*4.25073965847863e-23;
et113 = t16.*t30.*t72.*1.933613622435097e-22;
et114 = t17.*t30.*t72.*5.756958141897304e-23;
et115 = t18.*t30.*t72.*7.993777824483687e-23+t9.*t75.*t160;
et116 = t2.*t5.*t8.*t74.*3.46332667728404e-6+t4.*t5.*t8.*t74.*8.195215631096216e-7;
et117 = t2.*t8.*t9.*t74.*1.882396747564322e-6-t4.*t5.*t9.*t75.*8.376559107229145e-7;
et118 = t4.*t7.*t8.*t74.*1.253488085959302e-6+t5.*t6.*t8.*t74.*1.428633261714363e-5;
et119 = t5.*t8.*t9.*t71.*1.408936125616489e-6+t4.*t8.*t9.*t74.*4.454285918434201e-7;
et120 = t5.*t7.*t9.*t74.*(-4.287013106293682e-6)+t4.*t5.*t16.*t71.*5.4093083807222e-13;
et121 = t6.*t8.*t9.*t74.*7.764946411068142e-6-t4.*t9.*t16.*t71.*7.093613755211269e-13;
et122 = t5.*t8.*t16.*t71.*7.492102979241942e-7+t5.*t7.*t17.*t74.*1.378434177095879e-6;
et123 = t4.*t8.*t18.*t74.*8.376559107229145e-7-t8.*t9.*t16.*t71.*1.378434177095879e-6;
et124 = t2.*t3.*t30.*t72.*2.49373386785477e-22;
et125 = t7.*t9.*t17.*t74.*7.492102979241942e-7;
et126 = t2.*t4.*t30.*t72.*(-2.608176229845321e-22);
et127 = t3.*t4.*t30.*t72.*6.599207038311596e-23;
et128 = t3.*t5.*t30.*t72.*2.298746926034785e-23;
et129 = t3.*t6.*t30.*t72.*1.028673146211772e-21;
et130 = t4.*t5.*t30.*t72.*(-1.502780299100031e-21);
et131 = t2.*t8.*t30.*t72.*(-3.354896486533935e-22);
et132 = t4.*t6.*t30.*t72.*(-1.075880984259862e-21);
et133 = t4.*t7.*t30.*t72.*4.293116821085015e-23;
et134 = t8.*t16.*t18.*t71.*4.287013106293682e-6;
et135 = t3.*t9.*t30.*t72.*(-4.229348336668283e-23);
et136 = t4.*t8.*t30.*t72.*(-1.42236473075195e-22);
et137 = t5.*t7.*t30.*t72.*(-2.188339739859402e-29);
et138 = t4.*t9.*t30.*t72.*(-8.167952407966379e-22);
et139 = t5.*t9.*t30.*t72.*1.216145632129581e-22;
et140 = t6.*t8.*t30.*t72.*(-1.383905463411169e-21);
et141 = t7.*t17.*t18.*t74.*1.408936125616489e-6;
et142 = t7.*t8.*t30.*t72.*(-3.337571006928825e-23);
et143 = t7.*t9.*t30.*t72.*(-1.66874105402097e-29);
et144 = t5.*t16.*t30.*t72.*(-7.82072115054759e-23);
et145 = t5.*t17.*t30.*t72.*(-1.564144230109518e-22);
et146 = t7.*t17.*t30.*t72.*(-7.733879758902498e-23);
et147 = t9.*t16.*t30.*t72.*(-4.25073965847863e-23);
et148 = t9.*t17.*t30.*t72.*(-8.501479316957259e-23);
et149 = t16.*t17.*t30.*t72.*(-2.878479070948652e-23);
et150 = t16.*t18.*t30.*t72.*(-1.598755564896737e-22);
et151 = t17.*t18.*t30.*t72.*(-1.598755564896737e-22);
et152 = t4.*t5.*t7.*t8.*t74.*(-7.093613755211269e-13)+t4.*t5.*t8.*t9.*t74.*1.274380648825446e-6;
et153 = t4.*t7.*t8.*t9.*t74.*(-5.4093083807222e-13)-t5.*t8.*t9.*t16.*t71.*2.817872251232979e-6;
et154 = t2.*t3.*t5.*t30.*t72.*1.068001671898062e-22;
et155 = t5.*t7.*t9.*t17.*t74.*2.143506553146841e-6;
et156 = t2.*t4.*t5.*t30.*t72.*(-3.305064005090484e-22);
et157 = t3.*t4.*t5.*t30.*t72.*(-2.311271412620895e-23);
et158 = t2.*t4.*t7.*t30.*t72.*1.994589265414034e-22;
et159 = t2.*t3.*t9.*t30.*t72.*(-1.964962320751208e-22);
et160 = t3.*t5.*t6.*t30.*t72.*4.405540840394095e-22;
et161 = t2.*t4.*t9.*t30.*t72.*(-1.79637738896555e-22);
et162 = t4.*t5.*t6.*t30.*t72.*(-1.363349406435421e-21);
et163 = t3.*t4.*t9.*t30.*t72.*4.252391506801831e-23;
et164 = t3.*t5.*t8.*t30.*t72.*1.66874105402097e-29;
et165 = t2.*t7.*t8.*t30.*t72.*(-1.550641079758662e-22);
et166 = t4.*t5.*t8.*t30.*t72.*8.04930348521637e-29;
et167 = t4.*t6.*t7.*t30.*t72.*8.227744112962308e-22;
et168 = t3.*t6.*t9.*t30.*t72.*(-8.105532024608353e-22);
et169 = t3.*t7.*t8.*t30.*t72.*1.213683123456844e-22;
et170 = t4.*t6.*t9.*t30.*t72.*(-7.4101138229338e-22);
et171 = t4.*t7.*t8.*t30.*t72.*(-3.130253519639126e-23);
et172 = t3.*t8.*t9.*t30.*t72.*(-2.188339739859402e-29);
et173 = t5.*t7.*t8.*t30.*t72.*(-4.229348336668283e-23);
et174 = t4.*t8.*t9.*t30.*t72.*6.138079447808974e-29;
et175 = t6.*t7.*t8.*t30.*t72.*(-6.396443737329302e-22);
et176 = t7.*t8.*t9.*t30.*t72.*(-2.298746926034785e-23);
et177 = t3.*t4.*t18.*t30.*t72.*(-1.32251930673679e-22);
et178 = t4.*t8.*t16.*t30.*t72.*7.111823653759751e-23;
et179 = t5.*t7.*t17.*t30.*t72.*4.376679479718804e-29;
et180 = t5.*t9.*t16.*t30.*t72.*(-2.432291264259161e-22);
et181 = t5.*t9.*t17.*t30.*t72.*(-2.432291264259161e-22);
et182 = t7.*t9.*t17.*t30.*t72.*3.337482108041939e-29;
et183 = t5.*t16.*t17.*t30.*t72.*7.82072115054759e-23;
et184 = t9.*t16.*t17.*t30.*t72.*4.25073965847863e-23;
et185 = t16.*t17.*t18.*t30.*t72.*7.993777824483687e-23;
et186 = t3.*t4.*t5.*t7.*t30.*t72.*(-3.069039723904487e-29);
et187 = t3.*t4.*t5.*t9.*t30.*t72.*8.69297658713101e-23;
et188 = t2.*t5.*t7.*t8.*t30.*t72.*(-1.964962320751208e-22);
et189 = t3.*t4.*t7.*t9.*t30.*t72.*4.024651742608185e-29;
et190 = t3.*t5.*t7.*t8.*t30.*t72.*(-4.25073965847863e-23);
et191 = t4.*t5.*t7.*t8.*t30.*t72.*8.504783013603662e-23;
et192 = t2.*t7.*t8.*t9.*t30.*t72.*(-1.068001671898062e-22);
et193 = t5.*t6.*t7.*t8.*t30.*t72.*(-8.105532024608353e-22);
et194 = t3.*t7.*t8.*t9.*t30.*t72.*7.82072115054759e-23;
et195 = t4.*t7.*t8.*t9.*t30.*t72.*4.62254282524179e-23;
et196 = t6.*t7.*t8.*t9.*t30.*t72.*(-4.405540840394095e-22);
et197 = t4.*t5.*t8.*t16.*t30.*t72.*(-4.024651742608185e-29);
et198 = t3.*t7.*t8.*t18.*t30.*t72.*(-2.432291264259161e-22);
et199 = t4.*t7.*t8.*t18.*t30.*t72.*8.69297658713101e-23;
et200 = t4.*t8.*t9.*t16.*t30.*t72.*(-3.069039723904487e-29);
et201 = t5.*t9.*t16.*t17.*t30.*t72.*1.216145632129581e-22;
et202 = t3.*t5.*t7.*t8.*t9.*t30.*t72.*1.598755564896737e-22;
et203 = t4.*t5.*t7.*t8.*t9.*t30.*t72.*1.32251930673679e-22;
et204 = -t191+t334-t379-t397-t511+t521+t524-t671+t720+t773+t786-t816-t821+t923+t926+t931-t962.*3.383302988283333e-6-t963.*1.246862701090643e-6-t984-t1077+t1082+t1184+t1235;
et205 = t2.*t8.*(-7.30081420113316e-6);
et206 = t6.*t8.*1.769880715106441e-6+t9.*(t529-t967).*3.383302988283333e-6;
et207 = t2.*t4.*t5.*(-7.662598700988556e-13);
et208 = t2.*t4.*t7.*(-1.22799597575967e-5);
et209 = t2.*t3.*t9.*1.288848080425708e-12;
et210 = t4.*t5.*t6.*1.857585372652597e-13;
et211 = t4.*t6.*t7.*2.976937004352228e-6;
et212 = t3.*t6.*t9.*(-3.124456121473909e-13);
et213 = t2.*t4.*t75.*(-1.769880715106441e-6);
et214 = t2.*t8.*t71.*2.976937004352228e-6;
et215 = t2.*t9.*t74.*1.857585372652597e-13;
et216 = t4.*t6.*t75.*(-7.30081420113316e-6);
et217 = t6.*t8.*t71.*1.22799597575967e-5;
et218 = t6.*t9.*t74.*7.662598700988556e-13;
et219 = t2.*t5.*t7.*t8.*1.288848080425708e-12;
et220 = t5.*t6.*t7.*t8.*(-3.124456121473909e-13);
et221 = t2.*t4.*t5.*t71.*3.124456121473909e-13;
et222 = t4.*t5.*t6.*t71.*1.288848080425708e-12;
et223 = t2.*t5.*t8.*t75.*1.857585372652597e-13;
et224 = t5.*t6.*t8.*t75.*7.662598700988556e-13;
et225 = t2.*t3.*t4.*t30.*t72.*(-3.84506501891928e-22);
et226 = t3.*t4.*t6.*t30.*t72.*(-1.586101540900623e-21);
et227 = t2.*t7.*t9.*t30.*t72.*(-4.035603346078089e-29);
et228 = t6.*t7.*t9.*t30.*t72.*(-1.664699206432988e-28);
et229 = t2.*t3.*t5.*t8.*t30.*t72.*4.035603346078089e-29;
et230 = t3.*t5.*t6.*t8.*t30.*t72.*1.664699206432988e-28;
et231 = -t1417-t2.*t8.*3.96815841743287e-6;
et232 = t6.*t8.*9.619703863182361e-7;
et233 = t2.*t3.*t5.*(-1.288848080425708e-12);
et234 = t2.*t4.*t7.*(-6.674437170347525e-6);
et235 = t3.*t5.*t6.*3.124456121473909e-13;
et236 = t2.*t4.*t9.*(-7.662598700988556e-13);
et237 = t4.*t6.*t7.*1.618032907912407e-6;
et238 = t4.*t6.*t9.*1.857585372652597e-13;
et239 = t2.*t4.*t75.*(-9.619703863182361e-7);
et240 = t2.*t5.*t74.*(-1.857585372652597e-13);
et241 = t2.*t8.*t71.*1.618032907912407e-6;
et242 = t4.*t6.*t75.*(-3.96815841743287e-6);
et243 = t5.*t6.*t74.*(-7.662598700988556e-13);
et244 = t6.*t8.*t71.*6.674437170347525e-6;
et245 = t2.*t7.*t8.*t9.*1.288848080425708e-12;
et246 = t6.*t7.*t8.*t9.*(-3.124456121473909e-13);
et247 = t2.*t4.*t9.*t71.*3.124456121473909e-13;
et248 = t4.*t6.*t9.*t71.*1.288848080425708e-12;
et249 = t2.*t8.*t9.*t75.*1.857585372652597e-13;
et250 = t6.*t8.*t9.*t75.*7.662598700988556e-13;
et251 = t2.*t3.*t4.*t30.*t72.*(-2.089880210625419e-22);
et252 = t3.*t4.*t6.*t30.*t72.*(-8.620822290548326e-22);
et253 = t2.*t5.*t7.*t30.*t72.*4.035603346078089e-29;
et254 = t5.*t6.*t7.*t30.*t72.*1.664699206432988e-28;
et255 = t2.*t3.*t8.*t9.*t30.*t72.*4.035603346078089e-29;
et256 = t3.*t6.*t8.*t9.*t30.*t72.*1.664699206432988e-28;
et257 = t218+t232+t234+t246+t248+t251+t257+t258+t260+t261+t267+t268+t278+t282+t287+t289+t291+t292+t294+t295+t296+t298+t303+t305+t307+t315+t316+t319+t321+t322+t326+t327+t328+t329+t331+t332+t336+t337+t341+t343+t344+t345+t346+t347+t348+t349+t351+t353+t354+t365+t366+t374+t402+t442+t449+t451+t474+t486+t503+t505+t518+t522+t544+t553+t577+t582+t584+t585+t587+t590+t594+t597+t598+t600+t602+t604+t605+t606+t607+t611+t612+t615+t616+t617+t619+t620+t621+t622+t624+t625+t626+t627+t629+t633+t635+t636+t637+t638+t639+t640+t641+t642+t648+t650+t651+t652+t654+t657+t658+t662+t663+t664+t667+t673+t680+t699+t755+t756+t761+t770+t775+t780+t793+t811+t820+t823+t837+t856+t858+t862+t868+t869+t891+t901+t911+t916+t921+t930+t936+t945+t964+t968+t970+t974+t978+t999+t1019+t1032+t1041+t1071+t1089+t1102+t1105+t1106+t1107+t1108+t1110+t1112+t1113+t1114+t1115+t1116+t1118+t1120+t1121+t1123+t1124+t1126+t1128+t1129+t1131+t1134+t1136+t1139+t1140+t1141+t1142+t1143+t1144+t1145+t1152+t1155+t1158+t1159+t1160+t1166+t1169+t1170+t1172+t1173+t1175+t1176+t1177+t1178+t1179+t1180+t1181+t1183+t1190+t1192;
et258 = t1194+t1195+t1197+t1199+t1200+t1201+t1202+t1204+3.626861556360138e-4;
et259 = t962.*(-1.40259855e-11)+t966.*7.26350610236655e-5;
et260 = t4.*t5.*(-1.134411489642894e-5);
et261 = t3.*t9.*1.908078613917869e-5;
et262 = t9.*t74.*6.367841787827598e-4+t9.*(t529-t967).*1.40259855e-11;
et263 = t5.*t7.*t8.*1.908078613917869e-5;
et264 = t4.*t5.*t71.*3.698217217635989e-4+t4.*t9.*t74.*4.36041e-5;
et265 = t5.*t8.*t75.*6.367841787827598e-4;
et266 = t8.*t30.*t72.*6.93158769201428e-21;
et267 = t7.*t9.*t30.*t72.*(-7.142096628897415e-20);
et268 = t8.*t9.*t30.*t72.*4.161153561678485e-21;
et269 = t3.*t5.*t8.*t30.*t72.*7.142096628897415e-20;
et270 = t4.*t7.*t9.*t30.*t72.*(-2.47393392290267e-21);
et271 = t8.*1.134411489642894e-5+t75.*4.36041e-5;
et272 = t4.*t7.*1.908078613917869e-5;
et273 = t4.*t75.*6.367841787827598e-4;
et274 = t8.*t71.*(-3.698217217635989e-4)+t35.*t946+t38.*t946+t5.*(t529-t967).*7.26350610236655e-5;
et275 = t9.*(t529-t967).*(-1.33637579258949e-4)+t3.*t30.*t72.*2.47393392290267e-21;
et276 = t3.*t4.*t30.*t72.*7.142096628897415e-20;
et277 = t963.*1.40259855e-11+t966.*1.33637579258949e-4;
et278 = t3.*t5.*1.908078613917869e-5;
et279 = t4.*t9.*1.134411489642894e-5;
et280 = t5.*t74.*6.367841787827598e-4+t5.*(t529-t967).*1.40259855e-11;
et281 = t7.*t8.*t9.*(-1.908078613917869e-5)+t4.*t5.*t74.*4.36041e-5;
et282 = t4.*t9.*t71.*(-3.698217217635989e-4);
et283 = t8.*t9.*t75.*(-6.367841787827598e-4);
et284 = t8.*t30.*t72.*1.275307801118396e-20;
et285 = t5.*t7.*t30.*t72.*(-7.142096628897415e-20);
et286 = t5.*t8.*t30.*t72.*4.161153561678485e-21-t4.*t5.*t7.*t30.*t72.*2.47393392290267e-21;
et287 = t3.*t8.*t9.*t30.*t72.*(-7.142096628897415e-20);
et288 = t74.*3.876686599935835e-7+t383+t385+t408+t416+t595+t623+t1035+t1037+t1040+t1168;
et289 = (-t1363+t1248.*(t963+t5.*(t529-t967))+(t1251.*t1349.*(t26-t27))./1.316403645856965e+67).*(et259+et260+et261+et262+et263+et264+et265+et266+et267+et268+et269+et270);
et290 = t4.*t74.*(-1.20079068641418e-5)-t8.*t71.*2.170136264005124e-9;
et291 = t7.*t74.*2.22401922077146e-6+t8.*t74.*5.475413853010983e-6;
et292 = t17.*t74.*(-7.452373505947646e-7);
et293 = t30.*t72.*(-1.401374717769559e-20)+t75.*t134+t121.*t1420-t356.*t1417;
et294 = -t357.*t1416-(t1277-t1351+(t1251.*t1297.*(t26-t27))./1.316403645856965e+67).*(et271+et272+et273+et274+et275+et276);
et295 = (t1328+(t47.*t1251.*(t1292+t5.*(t647-t1222)))./1.316403645856965e+67+(t1251.*t1350.*(t26-t27))./1.316403645856965e+67).*(et277+et278+et279+et280+et281+et282+et283+et284+et285+et286+et287);
et296 = t4.*t8.*t74.*(-8.531618370996951e-7)+t8.*t16.*t71.*4.340272528010248e-9;
et297 = t7.*t17.*t74.*(-1.435017073119793e-6);
et298 = t4.*t30.*t72.*(-6.955757424542711e-22);
et299 = t7.*t30.*t72.*3.845355707634627e-23;
et300 = t8.*t30.*t72.*(-1.525438799069791e-21);
et301 = t16.*t30.*t72.*1.261825515365316e-22;
et302 = t17.*t30.*t72.*1.628350277673685e-22+t4.*t7.*t8.*t74.*1.253488230633412e-6;
et303 = t3.*t4.*t30.*t72.*(-1.338949537235126e-25);
et304 = t4.*t7.*t30.*t72.*4.293117264977958e-23;
et305 = t4.*t8.*t30.*t72.*(-1.422364894917333e-22);
et306 = t7.*t8.*t30.*t72.*(-1.957592943650879e-23);
et307 = t7.*t17.*t30.*t72.*(-7.733880651525396e-23);
et308 = t16.*t17.*t30.*t72.*(-8.141751388368425e-23);
et309 = t3.*t7.*t8.*t30.*t72.*(-2.462508672736528e-25);
et310 = t4.*t7.*t8.*t30.*t72.*(-8.853893084262633e-23);
et311 = t4.*t8.*t16.*t30.*t72.*7.111824474586663e-23;
et312 = t4.*(-2.117495204325297e-7);
et313 = t8.*9.655440125097679e-8+t75.*2.659783725725934e-6+t687;
et314 = t966.*1.758766830582798e-8-t967.*2.524706033578261e-9;
et315 = t4.*t7.*1.624043742404524e-7;
et316 = t7.*t8.*3.561624112004214e-7;
et317 = t4.*t71.*6.903101118415674e-6;
et318 = t4.*t75.*5.419930569269819e-6;
et319 = t8.*t71.*(-3.147703918772038e-6);
et320 = t8.*t75.*1.18862287368685e-5;
et321 = t3.*t30.*t72.*1.509062034684317e-22+t4.*t30.*t72.*2.409335246872506e-25;
et322 = t3.*t4.*t30.*t72.*6.078930528964336e-22;
et323 = t3.*t8.*t30.*t72.*1.333145467812469e-21;
et324 = t8.*6.806468937857363e-8+t75.*2.616246e-7;
et325 = t962.*8.01825475553694e-7+t963.*4.35810366141993e-7;
et326 = t4.*t7.*1.144847168350722e-7;
et327 = t4.*t75.*3.820705072696559e-6;
et328 = t8.*t71.*(-2.218930330581593e-6)+t5.*t1416+t9.*t1417+t5.*(t529-t967).*4.35810366141993e-7;
et329 = t9.*(t529-t967).*(-8.01825475553694e-7)+t1344.*(et312+et313+et314+et315+et316+et317+et318+et319+et320+et321+et322+et323)+t3.*t30.*t72.*1.484360353741602e-23;
et330 = t3.*t4.*t30.*t72.*4.285257977338449e-22;
et331 = t1345-t2.*t4.*t5.*5.463144604697158e-2;
et332 = t2.*t3.*t9.*9.189001945180305e-2;
et333 = t4.*t5.*t6.*1.324388487819695e-2;
et334 = t3.*t6.*t9.*(-2.227619671697157e-2);
et335 = t2.*t9.*t74.*1.324388487819695e-2;
et336 = t6.*t9.*t74.*5.463144604697158e-2;
et337 = t2.*t5.*t7.*t8.*9.189001945180305e-2;
et338 = t5.*t6.*t7.*t8.*(-2.227619671697157e-2);
et339 = t2.*t4.*t5.*t71.*2.227619671697157e-2;
et340 = t4.*t5.*t6.*t71.*9.189001945180305e-2;
et341 = t2.*t5.*t8.*t75.*1.324388487819695e-2;
et342 = t5.*t6.*t8.*t75.*5.463144604697158e-2-t2.*t7.*t9.*t30.*t72.*2.877233365226343e-18;
et343 = t6.*t7.*t9.*t30.*t72.*(-1.186867907736671e-17)+t2.*t3.*t5.*t8.*t30.*t72.*2.877233365226343e-18;
et344 = t3.*t5.*t6.*t8.*t30.*t72.*1.186867907736671e-17;
et345 = t1346-t2.*t3.*t5.*9.189001945180305e-2;
et346 = t3.*t5.*t6.*2.227619671697157e-2;
et347 = t2.*t4.*t9.*(-5.463144604697158e-2);
et348 = t4.*t6.*t9.*1.324388487819695e-2;
et349 = t2.*t5.*t74.*(-1.324388487819695e-2);
et350 = t5.*t6.*t74.*(-5.463144604697158e-2);
et351 = t2.*t7.*t8.*t9.*9.189001945180305e-2;
et352 = t6.*t7.*t8.*t9.*(-2.227619671697157e-2);
et353 = t2.*t4.*t9.*t71.*2.227619671697157e-2;
et354 = t4.*t6.*t9.*t71.*9.189001945180305e-2;
et355 = t2.*t8.*t9.*t75.*1.324388487819695e-2;
et356 = t6.*t8.*t9.*t75.*5.463144604697158e-2+t2.*t5.*t7.*t30.*t72.*2.877233365226343e-18;
et357 = t5.*t6.*t7.*t30.*t72.*1.186867907736671e-17+t2.*t3.*t8.*t9.*t30.*t72.*2.877233365226343e-18;
et358 = t3.*t6.*t8.*t9.*t30.*t72.*1.186867907736671e-17;
et359 = t1273-t2.*t4.*5.463144604697158e-2;
et360 = t4.*t6.*1.324388487819695e-2;
et361 = t2.*t7.*t8.*9.189001945180305e-2;
et362 = t6.*t7.*t8.*(-2.227619671697157e-2);
et363 = t2.*t4.*t71.*2.227619671697157e-2;
et364 = t4.*t6.*t71.*9.189001945180305e-2;
et365 = t2.*t8.*t75.*1.324388487819695e-2;
et366 = t6.*t8.*t75.*5.463144604697158e-2+t2.*t3.*t8.*t30.*t72.*2.877233365226343e-18;
et367 = t3.*t6.*t8.*t30.*t72.*1.186867907736671e-17;
et368 = t1247+t2.*t3.*9.189001945180305e-2;
et369 = t3.*t6.*(-2.227619671697157e-2);
et370 = t2.*t74.*1.324388487819695e-2+t6.*t74.*5.463144604697158e-2;
et371 = t2.*t7.*t30.*t72.*(-2.877233365226343e-18)-t6.*t7.*t30.*t72.*1.186867907736671e-17;
et372 = t380+t408+t579+t583+t586+t588+t591+t603+t623+t971+t1040+t1130+t1138+t1147+t1154+t1198+t1276+t1287+t1288+t1430+t1432+t1435-t1206.*(t196+t200+t217+t219+t566+t568+t569+t570+t670+t672+t1274)-t1415.*(t196+t200+t217+t219+t566+t568+t569+t570+t670+t672+t1283)+t1422.*(et331+et332+et333+et334+et335+et336+et337+et338+et339+et340+et341+et342+et343+et344)-t1421.*(et345+et346+et347+et348+et349+et350+et351+et352+et353+et354+et355+et356+et357+et358)+t2.*t75.*4.3770347702589e-6;
et373 = t6.*t75.*1.805540754063641e-5-t1207.*(et359+et360+et361+et362+et363+et364+et365+et366+et367)+t1219.*(et368+et369+et370+et371);
et374 = t2.*t30.*t72.*(-2.751435409876806e-21);
et375 = t6.*t30.*t72.*(-1.134975851337029e-20);
et376 = t2.*t3.*t30.*t72.*2.483366197185125e-22;
et377 = t3.*t6.*t30.*t72.*1.024396449109444e-21;
et378 = t3.*(-2.844856587289647e-6);
et379 = t4.*8.940013971103833e-6;
et380 = t5.*4.188040994443703e-7;
et381 = t7.*6.474095421643823e-7;
et382 = t8.*1.149953792156111e-5;
et383 = t9.*2.276295446893622e-7;
et384 = t16.*(-2.929443421869778e-6);
et385 = t17.*(-2.81948171692439e-7);
et386 = t18.*(-1.211065105878372e-6);
et387 = t19.*1.250511956078399e-9;
et388 = t20.*3.483029800032151e-7;
et389 = t21.*(-9.212362233958261e-7);
et390 = t3.*t4.*1.093188572509221e-6;
et391 = t3.*t5.*(-3.660776353481749e-6);
et392 = t4.*t5.*1.132872773043163e-5;
et393 = t3.*t8.*(-1.545129867076994e-8);
et394 = t4.*t7.*(-6.836829388815001e-6);
et395 = t3.*t9.*6.735277470591094e-6;
et396 = t5.*t7.*(-3.625084017661248e-13);
et397 = t4.*t9.*6.157420948384101e-6;
et398 = t7.*t8.*5.315113587256377e-6;
et399 = t7.*t9.*(-2.764345231392299e-13);
et400 = t5.*t16.*1.184846851663018e-6;
et401 = t5.*t17.*7.660427522186475e-7;
et402 = t7.*t17.*(-1.281152254279884e-6);
et403 = t9.*t16.*6.439911875946239e-7;
et404 = t9.*t17.*4.163616429052617e-7;
et405 = t16.*t17.*4.360923755161119e-7;
et406 = t16.*t18.*2.422130211756745e-6;
et407 = t17.*t18.*7.829937223708732e-7;
et408 = t3.*t4.*t5.*(-3.828725908394669e-7);
et409 = t3.*t4.*t7.*(-2.598906377458728e-8);
et410 = t3.*t4.*t9.*7.044279371874937e-7;
et411 = t3.*t5.*t8.*2.764345231392299e-13;
et412 = t4.*t5.*t8.*(-3.94216241479634e-13);
et413 = t3.*t7.*t8.*(-1.838741722230682e-6);
et414 = t4.*t7.*t8.*(-5.185406908527248e-7);
et415 = t3.*t8.*t9.*(-3.625084017661248e-13);
et416 = t5.*t7.*t8.*6.735277470591094e-6;
et417 = t4.*t8.*t9.*(-3.006136635626675e-13);
et418 = t7.*t8.*t9.*3.660776353481749e-6;
et419 = t3.*t4.*t18.*(-2.190813206274814e-6);
et420 = t4.*t8.*t16.*(-1.077448192248847e-6);
et421 = t5.*t7.*t17.*7.250168035322496e-13;
et422 = t5.*t9.*t16.*3.684944893583304e-6;
et423 = t5.*t9.*t17.*1.191219491402018e-6;
et424 = t7.*t9.*t17.*5.528690462784599e-13;
et425 = t5.*t16.*t17.*(-1.184846851663018e-6);
et426 = t9.*t16.*t17.*(-6.439911875946239e-7);
et427 = t16.*t17.*t18.*(-1.211065105878372e-6);
et428 = t3.*t4.*t5.*t7.*4.649624995570082e-13;
et429 = t3.*t4.*t5.*t9.*1.440030993265091e-6;
et430 = t3.*t4.*t7.*t9.*(-6.097386487095885e-13);
et431 = t3.*t5.*t7.*t8.*6.439911875946239e-7;
et432 = t4.*t5.*t7.*t8.*1.408855874374987e-6;
et433 = t3.*t7.*t8.*t9.*(-1.184846851663018e-6);
et434 = t4.*t7.*t8.*t9.*7.657451816789338e-7;
et435 = t4.*t5.*t8.*t16.*6.097386487095885e-13;
et436 = t3.*t7.*t8.*t18.*3.684944893583304e-6;
et437 = t4.*t7.*t8.*t18.*1.440030993265091e-6;
et438 = t4.*t8.*t9.*t16.*4.649624995570082e-13;
et439 = t5.*t9.*t16.*t17.*(-1.842472446791652e-6);
et440 = t3.*t5.*t7.*t8.*t9.*(-2.422130211756745e-6);
et441 = t4.*t5.*t7.*t8.*t9.*2.190813206274814e-6;
et442 = 8.99453681175877e-5;
et443 = t5.*8.195215631096216e-7+t7.*6.334299027523179e-7;
et444 = t9.*4.454285918434201e-7+t17.*3.016314764575132e-7+t141+t154+t163+t171+t180+t184+t233+t255+t262+t273+t288+t302+t362;
et445 = t3.*t4.*1.069583140309415e-6-t5.*t7.*3.546806877605634e-13;
et446 = t7.*t9.*(-2.7046541903611e-13)-t5.*t17.*8.195215631096216e-7;
et447 = t7.*t17.*(-1.253488085959302e-6)-t9.*t17.*4.454285918434201e-7;
et448 = t17.*t18.*(-8.376559107229145e-7)+t4.*t5.*t8.*4.217371804444381e-13;
et449 = t4.*t7.*t8.*(-5.073437414621283e-7)+t4.*t8.*t9.*3.216000396080637e-13;
et450 = t3.*t4.*t18.*(-2.143506553146841e-6)+t5.*t7.*t17.*7.093613755211269e-13;
et451 = t5.*t9.*t17.*(-1.274380648825446e-6)+t7.*t9.*t17.*5.4093083807222e-13;
et452 = t3.*t4.*t5.*t9.*1.408936125616489e-6+t4.*t5.*t7.*t8.*1.378434177095879e-6;
et453 = t4.*t7.*t8.*t9.*7.492102979241942e-7+t4.*t7.*t8.*t18.*1.408936125616489e-6;
et454 = t4.*t5.*t7.*t8.*t9.*2.143506553146841e-6+4.675266403474358e-6;
et455 = t1277.*(-4.36041e-5)-t3.*t5.*6.892170885479394e-7+t4.*t5.*2.227142959217101e-7;
et456 = t3.*t9.*(-3.746051489620971e-7)-t4.*t9.*4.097607815548108e-7-t5.*t1427+t9.*t1428-t1272.*t1344;
et457 = t5.*t7.*t8.*(-3.746051489620971e-7)+t7.*t8.*t9.*6.892170885479394e-7;
et458 = t47.*t1251.*t1290.*3.312365484343079e-72;
et459 = t1251.*t1297.*(t26-t27).*(-3.312365484343079e-72);
et460 = t90+t119+t150+t161-t168+t169-t172-t177+t1334-t1368+t1248.*(t963+t5.*(t529-t967)).*7.26350610236655e-5+t47.*t1251.*(t1292+t5.*(t647-t1222)).*1.015171749786156e-71;
et461 = t1251.*t1349.*(t26-t27).*5.517689141340903e-72;
et462 = t1251.*t1350.*(t26-t27).*1.015171749786156e-71;
et463 = t7.*4.434404699592312e-7;
et464 = t74.*1.343796452840321e-8;
et465 = t75.*8.307571936196077e-6+t391+t736.*(t963+t5.*(t529-t967));
et466 = t1345.*(t8.*7.26350610236655e-5+t4.*t9.*1.40259855e-11+t8.*t9.*4.36041e-5);
et467 = t30.*t72.*3.910962551211394e-22+t181.*t946+t4.*t1274.*7.051078772420001e-7+t8.*t1273.*7.051078772420001e-7-t712.*t1265+t1090.*t1208;
et468 = (t4.*2.257319918256733e-6-t8.*7.291452964015446e-7).*(t529-t967);
et469 = -t1346.*(t8.*1.33637579258949e-4+t4.*t5.*1.40259855e-11+t5.*t8.*4.36041e-5);
et470 = -t1208.*(t4.*7.291452964015446e-7-t8.*5.878412210495409e-7)+t1283.*(t4.*t5.*7.26350610236655e-5-t4.*t9.*1.33637579258949e-4);
et471 = -t1247.*(t4.*1.35652529206996e-4-t8.*6.185538795558e-5);
et472 = t3.*t30.*t72.*1.291537098619388e-21;
et473 = t7.*t30.*t72.*(-1.670883952997876e-24);
et474 = t5.*4.097607815548108e-7+t7.*6.685859772666872e-9;
et475 = t9.*2.227142959217101e-7-t14.*5.859823945197205e-8;
et476 = t15.*(-2.094139776807286e-7)-t21.*3.185951622063616e-7+t141+t154+t163+t171+t180+t184+t233+t255+t262+t273+t288+t302+t362;
et477 = t3.*t4.*(-2.170136264005124e-9)-t5.*t14.*4.097607815548108e-7;
et478 = t7.*t14.*(-6.267440429796511e-7)-t9.*t14.*2.227142959217101e-7;
et479 = t5.*t20.*2.10868590222219e-13+t7.*t20.*9.856216067305823e-8;
et480 = t9.*t20.*1.608000198040319e-13-t14.*t15.*2.094139776807286e-7;
et481 = t14.*t21.*(-3.185951622063616e-7)-t3.*t4.*t15.*1.07175327657342e-6;
et482 = t5.*t7.*t14.*3.546806877605634e-13+t3.*t4.*t21.*7.044680628082447e-7;
et483 = t7.*t9.*t14.*2.7046541903611e-13+t5.*t7.*t20.*6.892170885479394e-7;
et484 = t7.*t9.*t20.*3.746051489620971e-7+t7.*t15.*t20.*3.522340314041224e-7;
et485 = t7.*t20.*t21.*5.358766382867102e-7+4.616668164022386e-6;
et486 = t5.*1.603650951107388e-6+t9.*8.71620732283986e-7+t17.*5.902365793397849e-7-t20.*7.291452122456316e-7;
et487 = t5.*t17.*(-1.603650951107388e-6)-t9.*t17.*8.71620732283986e-7-t17.*t18.*1.639136489385872e-6+t4.*t5.*t8.*8.252610559395431e-13;
et488 = t4.*t8.*t9.*6.293113355513489e-13-t5.*t9.*t17.*2.493725402181286e-6+9.148624944245897e-6;
et489 = t953.*3.835762748795343e-73;
et490 = t1214.*3.835762748795343e-73;
et491 = t1216.*3.835762748795343e-73;
et492 = t953.*2.672078334207073e-72;
et493 = t1214.*2.672078334207073e-72;
et494 = t1216.*2.672078334207073e-72;
et495 = t953.*2.060956449549905e-68;
et496 = t1214.*2.060956449549905e-68;
et497 = t1216.*2.060956449549905e-68;
et498 = t953.*9.397632428359433e-69;
et499 = t1214.*9.397632428359433e-69;
et500 = t1216.*9.397632428359433e-69;
et501 = t368.*(t963+t5.*(t529-t967))-t5.*t1345.*1.40259855e-11-t9.*t1346.*1.40259855e-11-t186.*t1208+t364.*t1265+t355.*t1283+t946.*t1343+(t529-t8.*t74+t8.*t528).*(et489+et490+et491);
et502 = (et492+et493+et494).*(t530+t4.*t74-t4.*t7.*t30.*t72.*5.673626844500105e-17)+t1273.*(et495+et496+et497)+t1274.*(et498+et499+et500);
et503 = t9.*(t1328+(t47.*t1251.*(t1292+t5.*(t647-t1222)))./1.316403645856965e+67+(t1251.*t1350.*(t26-t27))./1.316403645856965e+67);
et504 = 1.40259855e-11;
et505 = -t101+t102+t134+t149-t153-t237-t240-t5.*(-t1363+t1248.*(t963+t5.*(t529-t967))+(t1251.*t1349.*(t26-t27))./1.316403645856965e+67).*1.40259855e-11+et503.*et504-t121.*t186-t357.*t364-t356.*t368;
et506 = -t355.*(t1277-t1351+(t1251.*t1297.*(t26-t27))./1.316403645856965e+67);
et507 = t953./6.582018229284824e+63+t1214./6.582018229284824e+63;
et508 = t1216./6.582018229284824e+63;
et509 = t227+t241+t386+t394+t395+t404+t405+t415+t424+t427+t441+t447+t448+t455+t458+t465+t471+t479+t496+t501+t668+t695+t702+t711+t730+t767+t779+t796+t801+t814+t829+t833+t841+t843+t845+t852+t854+t860+t867+t877+t886+t890+t905+t983+t993+t1001+t1007+t1010+t1028+t1029+t1030+t1036+t1038+t1050+t1058+t4.*t74.*4.20092050615074e-6-t5.*t75.*3.146556677756745e-13+t62.*t75+t8.*t717+t8.*t766;
et510 = t5.*t8.*t74.*(-4.126305279697715e-13)-t8.*t9.*t74.*3.146556677756745e-13-t3.*t5.*t30.*t72.*1.785238843466173e-29;
et511 = t4.*t5.*t30.*t72.*3.937746659416635e-29-t4.*t7.*t30.*t72.*2.383445535530781e-22;
et512 = t3.*t9.*t30.*t72.*2.341111640349547e-29+t4.*t9.*t30.*t72.*3.002769355787804e-29;
et513 = t1425.*(t1328+(t47.*t1251.*(t1292+t5.*(t647-t1222)))./1.316403645856965e+67+(t1251.*t1350.*(t26-t27))./1.316403645856965e+67)+t121.*t1439-t356.*t1438;
et514 = -t1436.*(t1277-t1351+(t1251.*t1297.*(t26-t27))./1.316403645856965e+67)-t357.*(-t1240+t1299+t1308+t1326+t1332+t1395+t1397+t1406+t1408);
et515 = (-t1363+t1248.*(t963+t5.*(t529-t967))+(t1251.*t1349.*(t26-t27))./1.316403645856965e+67).*(t1231-t1311+t1318+t1322-t1412+t1290.*(t1292+t5.*(t647-t1222)).*1.40259855e-11);
et516 = t1284.*8.01825475553694e-7+t1286.*4.35810366141993e-7+t1388.*4.35810366141993e-7+t1390.*4.35810366141993e-7;
et517 = t1391.*8.01825475553694e-7-t1290.*(t1292+t5.*(t647-t1222)).*8.01825475553694e-7+t9.*t1438+t5.*(-t1240+t1299+t1308+t1326+t1332+t1395+t1397+t1406+t1408);
mt1 = [et10+et11+et12+et13+et14+et15+et16+et17+et18+et19+et20+et21+et22+et23+et24+et25+et26+et27+et28+et29+et30+et31+et32+et33+et34+et35+et36+et37+et38+et39+et40+et41+et42+et43+et44+et45+et46+et47+et48+et49+et50+et51+et52+et53+et54+et55+et56+et57+et58+et59+et60+et61+et62+et63+et64+et65+et66+et67+et68+et69+et70+et71+et72+et73+et74+et75+et76+et77+et78+et79+et80+et81,t1442,et372+et373+et374+et375+et376+et377,t1441,t1440,et509+et510+et511+et512,t1442,et257+et258,t380+t408+t579+t586+t623+t971+t1040+t1130+t1154+t1198+t1276+t1287+t1288+t1430+t1432+t1435+t1219.*t1247-t1206.*t1274-t1207.*t1273-t1283.*t1415+t1345.*t1422-t1346.*t1421,et463+et464+et465+et466+et467+et468+et469+et470+et471+et472+et473,et501+et502];
mt2 = [t1438.*(t963+t5.*(t529-t967))+t1208.*t1439+t1283.*t1436-t1346.*t1425+t1265.*(-t1240+t1299+t1308+t1326+t1332+t1395+t1397+t1406+t1408)+t1345.*(t1231-t1311+t1318+t1322-t1412+t1290.*(t1292+t5.*(t647-t1222)).*1.40259855e-11)];
mt3 = [et82+et83+et84+et85+et86+et87+et88+et89+et90+et91+et92+et93+et94+et95+et96+et97+et98+et99+et100+et101+et102+et103+et104+et105+et106+et107+et108+et109+et110+et111+et112+et113+et114+et115+et116+et117+et118+et119+et120+et121+et122+et123+et124+et125+et126+et127+et128+et129+et130+et131+et132+et133+et134+et135+et136+et137+et138+et139+et140+et141+et142+et143+et144+et145+et146+et147+et148+et149+et150+et151+et152+et153+et154+et155+et156+et157+et158+et159+et160+et161+et162+et163+et164+et165+et166+et167+et168+et169+et170+et171+et172+et173+et174+et175+et176+et177+et178+et179+et180+et181+et182+et183+et184+et185+et186+et187+et188+et189+et190+et191+et192+et193+et194+et195+et196+et197+et198+et199+et200+et201+et202+et203,et288+et289+et290+et291+et292+et293+et294+et295+et296+et297+et298+et299+et300+et301+et302+et303+et304+et305+et306+et307+et308+et309+et310+et311];
mt4 = [et378+et379+et380+et381+et382+et383+et384+et385+et386+et387+et388+et389+et390+et391+et392+et393+et394+et395+et396+et397+et398+et399+et400+et401+et402+et403+et404+et405+et406+et407+et408+et409+et410+et411+et412+et413+et414+et415+et416+et417+et418+et419+et420+et421+et422+et423+et424+et425+et426+et427+et428+et429+et430+et431+et432+et433+et434+et435+et436+et437+et438+et439+et440+et441+et442,et474+et475+et476+et477+et478+et479+et480+et481+et482+et483+et484+et485,et505+et506,et513+et514+et515,t1441,t213+t228+t239+t243+t244+t250+t256+t259+t265+t266+t279+t293+t299+t304+t313+t314+t323+t359+t391+t409+t419+t425+t461+t463+t476+t548+t679+t689+t696+t701+t707+t714+t717+t718+t721+t725+t731+t734+t739+t741+t744+t745+t747+t748+t753+t758+t759+t766+t771+t772+t789+t791+t828+t840+t861+t863+t903+t906+t915+t918+t920+t922+t961+t1000+t1022+t1039+t1043+t1065+t1073+t1078+t1100,et443+et444+et445+et446+et447+et448+et449+et450+et451+et452+et453+et454,et486+et487+et488,t181-t8.*t186+t4.*t5.*t368-t4.*t9.*t364];
mt5 = [t8.*t1439-t4.*t9.*(-t1240+t1299+t1308+t1326+t1332+t1395+t1397+t1406+t1408)+t8.*t9.*(t1231-t1311+t1318+t1322-t1412+t1290.*(t1292+t5.*(t647-t1222)).*1.40259855e-11).*(3.0./5.0e+2)+t5.*t8.*t1425.*(3.0./5.0e+2)+t4.*t5.*t1438,t1440,et324+et325+et326+et327+et328+et329+et330,et455+et456+et457+et458+et459];
mt6 = [t4.*t5.*4.35810366141993e-7-t4.*t9.*8.01825475553694e-7-t5.*t712+t9.*t736+t181.*t1344];
mt7 = [t5.*8.01825475553694e-7+t9.*4.35810366141993e-7+t1343.*(et507+et508)+t5.*t364+t9.*t368+2.616246e-7,et516+et517];
mt8 = [t1387.*(t395+t405+t415+t427+t447+t448+t455+t458+t471+t479+t496+t501+t767+t779+t796+t801+t829+t841+t843+t845+t852+t854+t877+t890+t983+t993+t1007+t1010+t1028+t1030+t1036+t1050+t1420)-t1423.*(et204+et205+et206+et207+et208+et209+et210+et211+et212+et213+et214+et215+et216+et217+et218+et219+et220+et221+et222+et223+et224+et225+et226+et227+et228+et229+et230)-t1424.*(et231+et232+et233+et234+et235+et236+et237+et238+et239+et240+et241+et242+et243+et244+et245+et246+et247+et248+et249+et250+et251+et252+et253+et254+et255+et256),t1387.*t1420+t1416.*t1423+t1417.*t1424,t1387.*(et460+et461+et462)-t1423.*t1427+t1424.*t1428,-t712.*t1423+t736.*t1424+t1090.*t1387,-t186.*t1387+t364.*t1423+t368.*t1424,t1387.*t1439+t1424.*t1438+t1423.*(-t1240+t1299+t1308+t1326+t1332+t1395+t1397+t1406+t1408)];
H = reshape([mt1,mt2,mt3,mt4,mt5,mt6,mt7,mt8],6,6);
end
